simulink model "Test1_1"  (R2021a)
settings: Solver=FixedStepAuto  StartTime=0  StopTime=0.2  FixedStep=0.2  RelTol=1e-3
libraries: spsDistributedParametersLineLib x46, spsThreePhaseSeriesRLCLoadLib x15, spsThreePhaseVIMeasurementLib x3, spsGroundLib x1, spsThreePhaseSourceLib x1, spsSeriesRLCBranchLib x1, spspowerguiLib x1
settings Model: Creator=Admin  LastModifiedBy=Admin

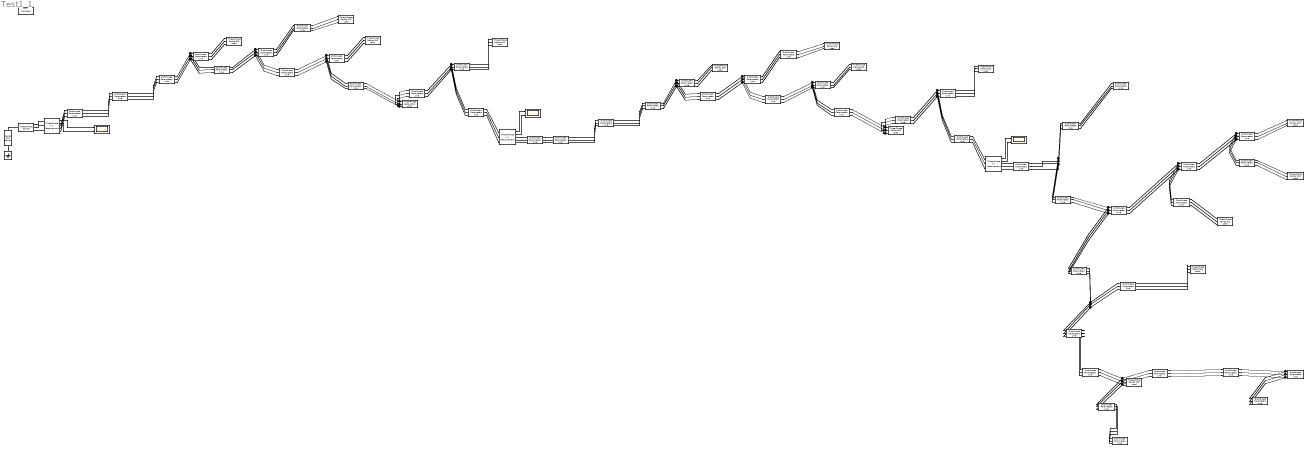
== system Test1_1 ==
  Ground : spsGroundLib/Ground  LConnTagsString=a
  Line 1 : spsDistributedParametersLineLib/Distributed Parameters Line  Phases=3  Length=0.24001  Frequency=50  Resistance=[0.646656091154803 0.0486237908083191 0.0486712220507153;0.0486237908083191 0.646561225344642 0.0486237934466192;0.0486712220507153 0.0486237934466192 0.646656091154803]  Inductance=[0.00282448912315926 0.00133270803418135 0.00132951476746136;0.00133270803418135 0.00282479813276775 0.00133799988507366;0.00132951476746136 0.00133799988507366 0.00282448912315926]  Capacitance=[7.89543174552926e-09 -1.85986777702161e-09 -1.7901190036642e-09;-1.85986777702161e-09 7.82540023894543e-09 -1.8957321828871e-09;-1.7901190036642e-09 -1.8957321828871e-09 7.91264394645417e-09]  x1=[156.806777459941 2289.04435554891 2292.85307010136;314.159265358979 314.159265358979 314.159265358979;1.01044698558813 -0.751410505261297 -2.32103514524067]  x2=[159.41925430945 1994.46757360395 1998.0250826666;314.159265358979 314.159265358979 314.159265358979;1.01620866542738 -0.846411494774192 -2.41545713049329]  x3=[6.24173255134266 1953.73927090339 1957.2720596961;314.159265358979 314.159265358979 314.159265358979;0.201344542731968 2.28105028050416 0.712425537947585]  x4=[6.05480721743813 1964.60242893867 1968.23812115216;314.159265358979 314.159265358979 314.159265358979;-2.97338155580937 -0.860183806246892 -2.42880992327048]  x5=1.1500013657538e-06  V1=ones(3,3)  V2=ones(3,3)  I1=ones(3,3)  I2=ones(3,3)  nHarmo=1  Measurements=None  Decoupling=off  VsMag0=0  VrMag0=0  VsAngle0=0  VrAngle0=0  IsMag0=0  IrMag0=0  IsAngle0=0  IrAngle0=0
      settings: SourceProductBaseCode=PS
  Line 10 : spsDistributedParametersLineLib/Distributed Parameters Line  Phases=3  Length=0.17  Frequency=50  Resistance=[0.646656091154803 0.0486237908083191 0.0486712220507153;0.0486237908083191 0.646561225344642 0.0486237934466192;0.0486712220507153 0.0486237934466192 0.646656091154803]  Inductance=[0.00282448912315926 0.00133270803418135 0.00132951476746136;0.00133270803418135 0.00282479813276775 0.00133799988507366;0.00132951476746136 0.00133799988507366 0.00282448912315926]  Capacitance=[7.89543174552926e-09 -1.85986777702161e-09 -1.7901190036642e-09;-1.85986777702161e-09 7.82540023894543e-09 -1.8957321828871e-09;-1.7901190036642e-09 -1.8957321828871e-09 7.91264394645417e-09]  x1=[137.717423229215 4738.81854218925 4741.80718996898;314.159265358979 314.159265358979 314.159265358979;0.961344854953636 -0.452365781969037 -2.02351010001284]  x2=[137.717927237638 4738.74941186832 4741.73816542518;314.159265358979 314.159265358979 314.159265358979;0.961345276145547 -0.452367573782606 -2.02351184606127]  x3=[0.121202473593997 11.5997833117508 11.6995568188445;314.159265358979 314.159265358979 314.159265358979;0.949832628337509 -0.42843606174828 -1.99977984923718]  x4=[0.119616166392622 12.521360958643 12.6220419925632;314.159265358979 314.159265358979 314.159265358979;0.972752580813695 -0.47473151222512 -2.04570347187694]  x5=8.14550361143895e-07  V1=ones(3,3)  V2=ones(3,3)  I1=ones(3,3)  I2=ones(3,3)  nHarmo=1  Measurements=None  Decoupling=off  VsMag0=0  VrMag0=0  VsAngle0=0  VrAngle0=0  IsMag0=0  IrMag0=0  IsAngle0=0  IrAngle0=0
      settings: SourceProductBaseCode=PS
  Line 11 : spsDistributedParametersLineLib/Distributed Parameters Line  Phases=3  Length=0.27999  Frequency=50  Resistance=[0.646656091154803 0.0486237908083191 0.0486712220507153;0.0486237908083191 0.646561225344642 0.0486237934466192;0.0486712220507153 0.0486237934466192 0.646656091154803]  Inductance=[0.00282448912315926 0.00133270803418135 0.00132951476746136;0.00133270803418135 0.00282479813276775 0.00133799988507366;0.00132951476746136 0.00133799988507366 0.00282448912315926]  Capacitance=[7.89543174552926e-09 -1.85986777702161e-09 -1.7901190036642e-09;-1.85986777702161e-09 7.82540023894543e-09 -1.8957321828871e-09;-1.7901190036642e-09 -1.8957321828871e-09 7.91264394645417e-09]  x1=[134.730981314477 5143.73431992549 5146.4499790882;314.159265358979 314.159265358979 314.159265358979;0.952121116671597 -0.431747792647745 -2.00297123761667]  x2=[137.717423229215 4738.81854218925 4741.80718996897;314.159265358979 314.159265358979 314.159265358979;0.96117928859628 -0.452497313565888 -2.02364175681846]  x3=[6.24015054861833 1949.40643992551 1952.88365407007;314.159265358979 314.159265358979 314.159265358979;0.19792740943073 2.27856091470476 0.70993208770443]  x4=[6.06948764855415 1972.37687159483 1976.07011587042;314.159265358979 314.159265358979 314.159265358979;-2.97066194767635 -0.857820676412098 -2.42644623491347]  x5=1.341564444804e-06  V1=ones(3,3)  V2=ones(3,3)  I1=ones(3,3)  I2=ones(3,3)  nHarmo=1  Measurements=None  Decoupling=off  VsMag0=0  VrMag0=0  VsAngle0=0  VrAngle0=0  IsMag0=0  IrMag0=0  IsAngle0=0  IrAngle0=0
      settings: SourceProductBaseCode=PS
  Line 12 : spsDistributedParametersLineLib/Distributed Parameters Line  Phases=3  Length=0.01  Frequency=50  Resistance=[0.646656091154803 0.0486237908083191 0.0486712220507153;0.0486237908083191 0.646561225344642 0.0486237934466192;0.0486712220507153 0.0486237934466192 0.646656091154803]  Inductance=[0.00282448912315926 0.00133270803418135 0.00132951476746136;0.00133270803418135 0.00282479813276775 0.00133799988507366;0.00132951476746136 0.00133799988507366 0.00282448912315926]  Capacitance=[7.89543174552926e-09 -1.85986777702161e-09 -1.7901190036642e-09;-1.85986777702161e-09 7.82540023894543e-09 -1.8957321828871e-09;-1.7901190036642e-09 -1.8957321828871e-09 7.91264394645417e-09]  x1=[134.624527579055 5158.23373249821 5160.93937939325;314.159265358979 314.159265358979 314.159265358979;0.952196584387825 -0.430744147583394 -2.00196980484842]  x2=[134.730981314477 5143.73431992549 5146.4499790882;314.159265358979 314.159265358979 314.159265358979;0.952527528716534 -0.431424924970376 -2.00264806259214]  x3=[6.24066120987054 1949.77580962925 1953.25644793354;314.159265358979 314.159265358979 314.159265358979;0.198319422837552 2.27887149292865 0.710242959177239]  x4=[6.07113450564641 1973.61885273018 1977.32373149217;314.159265358979 314.159265358979 314.159265358979;-2.96983216288509 -0.857163833200009 -2.42578877245703]  x5=4.79147271261115e-08  V1=ones(3,3)  V2=ones(3,3)  I1=ones(3,3)  I2=ones(3,3)  nHarmo=1  Measurements=None  Decoupling=off  VsMag0=0  VrMag0=0  VsAngle0=0  VrAngle0=0  IsMag0=0  IrMag0=0  IsAngle0=0  IrAngle0=0
      settings: SourceProductBaseCode=PS
  Line 13 : spsDistributedParametersLineLib/Distributed Parameters Line  Phases=3  Length=0.04  Frequency=50  Resistance=[0.646656091154803 0.0486237908083191 0.0486712220507153;0.0486237908083191 0.646561225344642 0.0486237934466192;0.0486712220507153 0.0486237934466192 0.646656091154803]  Inductance=[0.00282448912315926 0.00133270803418135 0.00132951476746136;0.00133270803418135 0.00282479813276775 0.00133799988507366;0.00132951476746136 0.00133799988507366 0.00282448912315926]  Capacitance=[7.89543174552926e-09 -1.85986777702161e-09 -1.7901190036642e-09;-1.85986777702161e-09 7.82540023894543e-09 -1.8957321828871e-09;-1.7901190036642e-09 -1.8957321828871e-09 7.91264394645417e-09]  x1=[134.198860362037 5216.25494933431 5218.9203856369;314.159265358979 314.159265358979 314.159265358979;0.950822400125934 -0.428094767615988 -1.9993303521305]  x2=[134.624527579055 5158.23373249821 5160.93937939325;314.159265358979 314.159265358979 314.159265358979;0.952151425821402 -0.430780023098491 -2.00200571451447]  x3=[6.24044022443603 1949.6120636545 1953.09117465905;314.159265358979 314.159265358979 314.159265358979;0.198214322239693 2.27878764327756 0.710159028664123]  x4=[6.07111576572209 1973.60352039945 1977.3082528197;314.159265358979 314.159265358979 314.159265358979;-2.96986211621341 -0.85718782340359 -2.42581278603856]  x5=1.91658908504446e-07  V1=ones(3,3)  V2=ones(3,3)  I1=ones(3,3)  I2=ones(3,3)  nHarmo=1  Measurements=None  Decoupling=off  VsMag0=0  VrMag0=0  VsAngle0=0  VrAngle0=0  IsMag0=0  IrMag0=0  IsAngle0=0  IrAngle0=0
      settings: SourceProductBaseCode=PS
  Line 2 : spsDistributedParametersLineLib/Distributed Parameters Line  Phases=3  Length=0.02  Frequency=50  Resistance=[0.646656091154803 0.0486237908083191 0.0486712220507153;0.0486237908083191 0.646561225344642 0.0486237934466192;0.0486712220507153 0.0486237934466192 0.646656091154803]  Inductance=[0.00282448912315926 0.00133270803418135 0.00132951476746136;0.00133270803418135 0.00282479813276775 0.00133799988507366;0.00132951476746136 0.00133799988507366 0.00282448912315926]  Capacitance=[7.89543174552926e-09 -1.85986777702161e-09 -1.7901190036642e-09;-1.85986777702161e-09 7.82540023894543e-09 -1.8957321828871e-09;-1.7901190036642e-09 -1.8957321828871e-09 7.91264394645417e-09]  x1=[156.806777459941 2289.04435554891 2292.85307010136;314.159265358979 314.159265358979 314.159265358979;1.01077816346141 -0.751147406192081 -2.32077179571977]  x2=[156.806785976177 2289.04321851652 2292.85193332345;314.159265358979 314.159265358979 314.159265358979;1.01077815828353 -0.751147536284466 -2.32077192407531]  x3=[0.13717054036225 5.75443719278579 5.80881227749304;314.159265358979 314.159265358979 314.159265358979;1.00918028356381 -0.745806305067407 -2.31547605369833]  x4=[0.137030436627376 5.89619014071261 5.95082798871036;314.159265358979 314.159265358979 314.159265358979;1.01234755059242 -0.756383856543157 -2.32596493554703]  x5=9.5829454252223e-08  V1=ones(3,3)  V2=ones(3,3)  I1=ones(3,3)  I2=ones(3,3)  nHarmo=1  Measurements=None  Decoupling=off  VsMag0=0  VrMag0=0  VsAngle0=0  VrAngle0=0  IsMag0=0  IrMag0=0  IsAngle0=0  IrAngle0=0
      settings: SourceProductBaseCode=PS
  Line 3 : spsDistributedParametersLineLib/Distributed Parameters Line  Phases=3  Length=0.5  Frequency=50  Resistance=[0.646656091154803 0.0486237908083191 0.0486712220507153;0.0486237908083191 0.646561225344642 0.0486237934466192;0.0486712220507153 0.0486237934466192 0.646656091154803]  Inductance=[0.00282448912315926 0.00133270803418135 0.00132951476746136;0.00133270803418135 0.00282479813276775 0.00133799988507366;0.00132951476746136 0.00133799988507366 0.00282448912315926]  Capacitance=[7.89543174552926e-09 -1.85986777702161e-09 -1.7901190036642e-09;-1.85986777702161e-09 7.82540023894543e-09 -1.8957321828871e-09;-1.7901190036642e-09 -1.8957321828871e-09 7.91264394645417e-09]  x1=[151.381670066741 2947.95085767605 2951.82529065523;314.159265358979 314.159265358979 314.159265358979;0.997415388913609 -0.617619917483095 -2.18800176165379]  x2=[156.806777459941 2289.04435554891 2292.85307010136;314.159265358979 314.159265358979 314.159265358979;1.01005562639866 -0.751721414433634 -2.32134635037653]  x3=[6.23941383066717 1951.93705204109 1955.45243536136;314.159265358979 314.159265358979 314.159265358979;0.200188858984882 2.28012943253653 0.711503799574193]  x4=[6.05546788002709 1965.0024474538 1968.64128594745;314.159265358979 314.159265358979 314.159265358979;-2.97342375138114 -0.860219461653461 -2.42884562437829]  x5=2.39573635630557e-06  V1=ones(3,3)  V2=ones(3,3)  I1=ones(3,3)  I2=ones(3,3)  nHarmo=1  Measurements=None  Decoupling=off  VsMag0=0  VrMag0=0  VsAngle0=0  VrAngle0=0  IsMag0=0  IrMag0=0  IsAngle0=0  IrAngle0=0
      settings: SourceProductBaseCode=PS
  Line 4 : spsDistributedParametersLineLib/Distributed Parameters Line  Phases=3  Length=0.23  Frequency=50  Resistance=[0.646656091154803 0.0486237908083191 0.0486712220507153;0.0486237908083191 0.646561225344642 0.0486237934466192;0.0486712220507153 0.0486237934466192 0.646656091154803]  Inductance=[0.00282448912315926 0.00133270803418135 0.00132951476746136;0.00133270803418135 0.00282479813276775 0.00133799988507366;0.00132951476746136 0.00133799988507366 0.00282448912315926]  Capacitance=[7.89543174552926e-09 -1.85986777702161e-09 -1.7901190036642e-09;-1.85986777702161e-09 7.82540023894543e-09 -1.8957321828871e-09;-1.7901190036642e-09 -1.8957321828871e-09 7.91264394645417e-09]  x1=[148.893866632266 3263.64496633825 3267.43134956967;314.159265358979 314.159265358979 314.159265358979;0.991698295023853 -0.574139543862195 -2.14474183596209]  x2=[151.381670066741 2947.95085767605 2951.82529065523;314.159265358979 314.159265358979 314.159265358979;0.997821816011403 -0.617297037847221 -2.18767857465937]  x3=[6.24075884536362 1952.25898948164 1955.77238425822;314.159265358979 314.159265358979 314.159265358979;0.200159169891873 2.2801199867809 0.711493977116933]  x4=[6.05971930332911 1967.50475507511 1971.16201304221;314.159265358979 314.159265358979 314.159265358979;-2.97234682394957 -0.859356129090504 -2.42798183096632]  x5=1.10203872390056e-06  V1=ones(3,3)  V2=ones(3,3)  I1=ones(3,3)  I2=ones(3,3)  nHarmo=1  Measurements=None  Decoupling=off  VsMag0=0  VrMag0=0  VsAngle0=0  VrAngle0=0  IsMag0=0  IrMag0=0  IsAngle0=0  IrAngle0=0
      settings: SourceProductBaseCode=PS
  Line 44 : spsDistributedParametersLineLib/Distributed Parameters Line  Phases=3  Length=1.1099  Frequency=50  Resistance=[0.502970710632245 0.0486237908083191 0.0486712220507153;0.0486237908083191 0.502875844822084 0.0486237934466192;0.0486712220507153 0.0486237934466192 0.502970710632245]  Inductance=[0.00286900545038753 0.00133270803418135 0.00132951476746136;0.00133270803418135 0.00286931445999602 0.00133799988507366;0.00132951476746136 0.00133799988507366 0.00286900545038753]  Capacitance=[8.11484299003193e-09 -1.94249816214699e-09 -1.86930692621136e-09;-1.94249816214699e-09 8.0425699231653e-09 -1.98049571960044e-09;-1.86930692621136e-09 -1.98049571960044e-09 8.13337738722527e-09]  x1=[176.041178073117 1994.09587758174 1997.08496491156;314.159265358979 314.159265358979 314.159265358979;0.937512580231571 -0.841595516654179 -2.41068590837705]  x2=[176.041429024076 1994.09774203895 1997.08683636866;314.159265358979 314.159265358979 314.159265358979;0.937512088108202 -0.841596394298114 -2.41068679358083]  x3=[0.154334056344399 5.07254983951833 5.11916023387305;314.159265358979 314.159265358979 314.159265358979;0.935823830196104 -0.84296342635579 -2.41205536081699]  x4=[0.15433405650098 5.0725498409922 5.11916023562135;314.159265358979 314.159265358979 314.159265358979;0.937512087880638 -0.84159639430282 -2.41068679356359]  x5=5.37467579168161e-06  V1=ones(3,3)  V2=ones(3,3)  I1=ones(3,3)  I2=ones(3,3)  nHarmo=1  Measurements=None  Decoupling=off  VsMag0=0  VrMag0=0  VsAngle0=0  VrAngle0=0  IsMag0=0  IrMag0=0  IsAngle0=0  IrAngle0=0
      settings: SourceProductBaseCode=PS
  Line 45 : spsDistributedParametersLineLib/Distributed Parameters Line  Phases=3  Length=0.03  Frequency=50  Resistance=[0.476003738225748 0.351747138225748 0.351747138225748;0.351747138225748 0.476003738225748 0.351747138225748;0.351747138225748 0.351747138225748 0.476003738225748]  Inductance=[0.000705954362986426 0.000459934243504405 0.000459934243504405;0.000459934243504405 0.000705954362986426 0.000459934243504405;0.000459934243504405 0.000459934243504405 0.000705954362986426]  Capacitance=[5.7561313269996e-07 -1.37543883484145e-07 -1.37543912800485e-07;-1.37543883484145e-07 5.75613027339387e-07 -1.37543875208088e-07;-1.37543912800485e-07 -1.37543875208088e-07 5.75613005057695e-07]  x1=[140.067507206974 1994.04557140135 1997.97862030497;314.159265358979 314.159265358979 314.159265358979;1.13103266143179 -0.764805817062905 -2.33393929024607]  x2=[140.067512372288 1994.04560306697 1997.97865212982;314.159265358979 314.159265358979 314.159265358979;1.13103254429501 -0.764805842557438 -2.33393931587598]  x3=[1.90359295650131 107.343811588221 107.55551404486;314.159265358979 314.159265358979 314.159265358979;1.13069546040223 -0.764995323142153 -2.33412939096158]  x4=[1.90368522741435 107.343794545186 107.555524609154;314.159265358979 314.159265358979 314.159265358979;1.13116138069285 -0.76474118135641 -2.33387406006431]  x5=6.63129528657629e-07  V1=ones(3,3)  V2=ones(3,3)  I1=ones(3,3)  I2=ones(3,3)  nHarmo=1  Measurements=None  Decoupling=off  VsMag0=0  VrMag0=0  VsAngle0=0  VrAngle0=0  IsMag0=0  IrMag0=0  IsAngle0=0  IrAngle0=0
      settings: SourceProductBaseCode=PS
  Line 46 : spsDistributedParametersLineLib/Distributed Parameters Line  Phases=3  Length=0.28002  Frequency=50  Resistance=[0.476003738225748 0.351747138225748 0.351747138225748;0.351747138225748 0.476003738225748 0.351747138225748;0.351747138225748 0.351747138225748 0.476003738225748]  Inductance=[0.000705954362986426 0.000459934243504405 0.000459934243504405;0.000459934243504405 0.000705954362986426 0.000459934243504405;0.000459934243504405 0.000459934243504405 0.000705954362986426]  Capacitance=[5.7561313269996e-07 -1.37543883484145e-07 -1.37543912800485e-07;-1.37543883484145e-07 5.75613027339387e-07 -1.37543875208088e-07;-1.37543912800485e-07 -1.37543875208088e-07 5.75613005057695e-07]  x1=[140.067507206974 1994.04557140135 1997.97862030497;314.159265358979 314.159265358979 314.159265358979;1.12929645349993 -0.765846222255273 -2.33497969535801]  x2=[140.067787182756 1994.04703476282 1997.98008719615;314.159265358979 314.159265358979 314.159265358979;1.12929162670007 -0.765847401848355 -2.33498087583294]  x3=[1.89789588728064 107.209321409248 107.420763113053;314.159265358979 314.159265358979 314.159265358979;1.12725437496433 -0.76705912034498 -2.33619301026011]  x4=[1.89796082095005 107.209309806491 107.420770208945;314.159265358979 314.159265358979 314.159265358979;1.12938694957278 -0.765800293242872 -2.33493335043468]  x5=6.18965102049031e-06  V1=ones(3,3)  V2=ones(3,3)  I1=ones(3,3)  I2=ones(3,3)  nHarmo=1  Measurements=None  Decoupling=off  VsMag0=0  VrMag0=0  VsAngle0=0  VrAngle0=0  IsMag0=0  IrMag0=0  IsAngle0=0  IrAngle0=0
      settings: SourceProductBaseCode=PS
  Line 47 : spsDistributedParametersLineLib/Distributed Parameters Line  Phases=3  Length=0.28002  Frequency=50  Resistance=[0.646656091154803 0.0486237908083191 0.0486712220507153;0.0486237908083191 0.646561225344642 0.0486237934466192;0.0486712220507153 0.0486237934466192 0.646656091154803]  Inductance=[0.00282448912315926 0.00133270803418135 0.00132951476746136;0.00133270803418135 0.00282479813276775 0.00133799988507366;0.00132951476746136 0.00133799988507366 0.00282448912315926]  Capacitance=[7.89543174552926e-09 -1.85986777702161e-09 -1.7901190036642e-09;-1.85986777702161e-09 7.82540023894543e-09 -1.8957321828871e-09;-1.7901190036642e-09 -1.8957321828871e-09 7.91264394645417e-09]  x1=[159.450836212371 1994.03630645724 1997.5930850958;314.159265358979 314.159265358979 314.159265358979;1.01609729305141 -0.846696591151605 -2.41574119338602]  x2=[159.450906639713 1994.03685996462 1997.59364061124;314.159265358979 314.159265358979 314.159265358979;1.01609710390738 -0.846696944332278 -2.4157415495164]  x3=[0.139394917805582 5.07298472412607 5.12105417855764;314.159265358979 314.159265358979 314.159265358979;1.01483976738527 -0.847693086082789 -2.41673856198392]  x4=[0.139394174108232 5.07298484806111 5.12105412073545;314.159265358979 314.159265358979 314.159265358979;1.01693310594968 -0.846035347146105 -2.41507939770091]  x5=1.34170818898537e-06  V1=ones(3,3)  V2=ones(3,3)  I1=ones(3,3)  I2=ones(3,3)  nHarmo=1  Measurements=None  Decoupling=off  VsMag0=0  VrMag0=0  VsAngle0=0  VrAngle0=0  IsMag0=0  IrMag0=0  IsAngle0=0  IrAngle0=0
      settings: SourceProductBaseCode=PS
  Line 48 : spsDistributedParametersLineLib/Distributed Parameters Line  Phases=3  Length=0.3  Frequency=50  Resistance=[0.80718830189013 0.0486237908083191 0.0486712220507153;0.0486237908083191 0.807093436079969 0.0486237934466192;0.0486712220507153 0.0486237934466192 0.80718830189013]  Inductance=[0.00279786707424938 0.00133270803418135 0.00132951476746136;0.00133270803418135 0.00279817608385787 0.00133799988507366;0.00132951476746136 0.00133799988507366 0.00279786707424938]  Capacitance=[7.73340098830622e-09 -1.79942827973291e-09 -1.73218055098733e-09;-1.79942827973291e-09 7.66505189233746e-09 -1.83375898618858e-09;-1.73218055098733e-09 -1.83375898618858e-09 7.749673531177e-09]  x1=[147.939133023316 1994.00252129492 1997.97662588148;314.159265358979 314.159265358979 314.159265358979;1.08434791512588 -0.850955285689131 -2.4199425962697]  x2=[147.939147884205 1994.00264447014 1997.97674951097;314.159265358979 314.159265358979 314.159265358979;1.08434786220581 -0.850955387187637 -2.41994269861345]  x3=[0.128901027196759 5.05947408132654 5.1081835056915;314.159265358979 314.159265358979 314.159265358979;1.08389966452075 -0.851306827100118 -2.42029443513027]  x4=[0.128901026894174 5.05947408128851 5.10818350470838;314.159265358979 314.159265358979 314.159265358979;1.08434786133197 -0.850955387242975 -2.41994269861003]  x5=1.42674452918375e-06  V1=ones(3,3)  V2=ones(3,3)  I1=ones(3,3)  I2=ones(3,3)  nHarmo=1  Measurements=None  Decoupling=off  VsMag0=0  VrMag0=0  VsAngle0=0  VrAngle0=0  IsMag0=0  IrMag0=0  IsAngle0=0  IrAngle0=0
      settings: SourceProductBaseCode=PS
  Line 49 : spsDistributedParametersLineLib/Distributed Parameters Line  Phases=3  Length=0.26  Frequency=50  Resistance=[0.646656091154803 0.0486237908083191 0.0486712220507153;0.0486237908083191 0.646561225344642 0.0486237934466192;0.0486712220507153 0.0486237934466192 0.646656091154803]  Inductance=[0.00282448912315926 0.00133270803418135 0.00132951476746136;0.00133270803418135 0.00282479813276775 0.00133799988507366;0.00132951476746136 0.00133799988507366 0.00282448912315926]  Capacitance=[7.89543174552926e-09 -1.85986777702161e-09 -1.7901190036642e-09;-1.85986777702161e-09 7.82540023894543e-09 -1.8957321828871e-09;-1.7901190036642e-09 -1.8957321828871e-09 7.91264394645417e-09]  x1=[159.450906639713 1994.03685996462 1997.59364061124;314.159265358979 314.159265358979 314.159265358979;1.01612723972403 -0.846673003405204 -2.41571758579925]  x2=[159.450918851672 1994.03695634835 1997.59373735104;314.159265358979 314.159265358979 314.159265358979;1.01612720669562 -0.8466730649035 -2.41571764781801]  x3=[0.139395866645988 5.07309981328857 5.12117114312411;314.159265358979 314.159265358979 314.159265358979;1.01573584725394 -0.846983955099221 -2.41602883408079]  x4=[0.139395866634972 5.07309981174401 5.12117114133114;314.159265358979 314.159265358979 314.159265358979;1.01612720842007 -0.846673065089804 -2.41571764765183]  x5=1.2457829052789e-06  V1=ones(3,3)  V2=ones(3,3)  I1=ones(3,3)  I2=ones(3,3)  nHarmo=1  Measurements=None  Decoupling=off  VsMag0=0  VrMag0=0  VsAngle0=0  VrAngle0=0  IsMag0=0  IrMag0=0  IsAngle0=0  IrAngle0=0
      settings: SourceProductBaseCode=PS
  Line 5 : spsDistributedParametersLineLib/Distributed Parameters Line  Phases=3  Length=1.62  Frequency=50  Resistance=[0.80718830189013 0.0486237908083191 0.0486712220507153;0.0486237908083191 0.807093436079969 0.0486237934466192;0.0486712220507153 0.0486237934466192 0.80718830189013]  Inductance=[0.00279786707424938 0.00133270803418135 0.00132951476746136;0.00133270803418135 0.00279817608385787 0.00133799988507366;0.00132951476746136 0.00133799988507366 0.00279786707424938]  Capacitance=[7.73340098830622e-09 -1.79942827973291e-09 -1.73218055098733e-09;-1.79942827973291e-09 7.66505189233746e-09 -1.83375898618858e-09;-1.73218055098733e-09 -1.83375898618858e-09 7.749673531177e-09]  x1=[125.888199100643 3263.65966141635 3267.79031196594;314.159265358979 314.159265358979 314.159265358979;1.07014406284904 -0.580039195774503 -2.15061989958838]  x2=[125.88865872902 3263.65855558813 3267.78922946379;314.159265358979 314.159265358979 314.159265358979;1.07014242225172 -0.580042000961513 -2.15062272408421]  x3=[0.109612775122241 8.2613178446553 8.33470841629561;314.159265358979 314.159265358979 314.159265358979;1.06747299264217 -0.58159829134088 -2.15218332448631]  x4=[0.109592728656291 8.26922562456906 8.34262765841689;314.159265358979 314.159265358979 314.159265358979;1.07039257279993 -0.580383016472921 -2.15096102526835]  x5=7.70442045759223e-06  V1=ones(3,3)  V2=ones(3,3)  I1=ones(3,3)  I2=ones(3,3)  nHarmo=1  Measurements=None  Decoupling=off  VsMag0=0  VrMag0=0  VsAngle0=0  VrAngle0=0  IsMag0=0  IrMag0=0  IsAngle0=0  IrAngle0=0
      settings: SourceProductBaseCode=PS
  Line 50 : spsDistributedParametersLineLib/Distributed Parameters Line  Phases=3  Length=0.02  Frequency=50  Resistance=[0.476003738225748 0.351747138225748 0.351747138225748;0.351747138225748 0.476003738225748 0.351747138225748;0.351747138225748 0.351747138225748 0.476003738225748]  Inductance=[0.000705954362986426 0.000459934243504405 0.000459934243504405;0.000459934243504405 0.000705954362986426 0.000459934243504405;0.000459934243504405 0.000459934243504405 0.000705954362986426]  Capacitance=[5.7561313269996e-07 -1.37543883484145e-07 -1.37543912800485e-07;-1.37543883484145e-07 5.75613027339387e-07 -1.37543875208088e-07;-1.37543912800485e-07 -1.37543875208088e-07 5.75613005057695e-07]  x1=[140.067461475806 1994.04572193785 1997.97877102815;314.159265358979 314.159265358979 314.159265358979;1.1311028945428 -0.764763926143592 -2.33389739917688]  x2=[140.067507206974 1994.04557140135 1997.97862030497;314.159265358979 314.159265358979 314.159265358979;1.13110210419364 -0.76476420418424 -2.33389767737062]  x3=[1.90379458359188 107.205560232195 107.416980727275;314.159265358979 314.159265358979 314.159265358979;1.12858679885131 -0.766052580413334 -2.33518706516769]  x4=[1.90395210493187 107.492988877227 107.705022727871;314.159265358979 314.159265358979 314.159265358979;1.13347910084245 -0.76356211258393 -2.33269457728375]  x5=4.42086352438419e-07  V1=ones(3,3)  V2=ones(3,3)  I1=ones(3,3)  I2=ones(3,3)  nHarmo=1  Measurements=None  Decoupling=off  VsMag0=0  VrMag0=0  VsAngle0=0  VrAngle0=0  IsMag0=0  IrMag0=0  IsAngle0=0  IrAngle0=0
      settings: SourceProductBaseCode=PS
  Line 51 : spsDistributedParametersLineLib/Distributed Parameters Line  Phases=3  Length=1.7101  Frequency=50  Resistance=[0.646656091154803 0.0486237908083191 0.0486712220507153;0.0486237908083191 0.646561225344642 0.0486237934466192;0.0486712220507153 0.0486237934466192 0.646656091154803]  Inductance=[0.00282448912315926 0.00133270803418135 0.00132951476746136;0.00133270803418135 0.00282479813276775 0.00133799988507366;0.00132951476746136 0.00133799988507366 0.00282448912315926]  Capacitance=[7.89543174552926e-09 -1.85986777702161e-09 -1.7901190036642e-09;-1.85986777702161e-09 7.82540023894543e-09 -1.8957321828871e-09;-1.7901190036642e-09 -1.8957321828871e-09 7.91264394645417e-09]  x1=[159.434216924154 1994.06687305595 1997.62429499923;314.159265358979 314.159265358979 314.159265358979;1.01397051629518 -0.848273829914017 -2.41732040176447]  x2=[159.450432897163 1994.03499301366 1997.59176799127;314.159265358979 314.159265358979 314.159265358979;1.01394953072372 -0.848405295765299 -2.4174515240815]  x3=[0.140424357868487 4.92335462242945 4.97106245663484;314.159265358979 314.159265358979 314.159265358979;0.976689775708697 -0.878406592183143 -2.44725440560169]  x4=[0.138339009885764 5.2101863624961 5.25832174536216;314.159265358979 314.159265358979 314.159265358979;1.04919801792014 -0.821918225205559 -2.39114198119224]  x5=8.19389748583632e-06  V1=ones(3,3)  V2=ones(3,3)  I1=ones(3,3)  I2=ones(3,3)  nHarmo=1  Measurements=None  Decoupling=off  VsMag0=0  VrMag0=0  VsAngle0=0  VrAngle0=0  IsMag0=0  IrMag0=0  IsAngle0=0  IrAngle0=0
      settings: SourceProductBaseCode=PS
  Line 52 : spsDistributedParametersLineLib/Distributed Parameters Line  Phases=3  Length=0.02  Frequency=50  Resistance=[0.646656091154803 0.0486237908083191 0.0486712220507153;0.0486237908083191 0.646561225344642 0.0486237934466192;0.0486712220507153 0.0486237934466192 0.646656091154803]  Inductance=[0.00282448912315926 0.00133270803418135 0.00132951476746136;0.00133270803418135 0.00282479813276775 0.00133799988507366;0.00132951476746136 0.00133799988507366 0.00282448912315926]  Capacitance=[7.89543174552926e-09 -1.85986777702161e-09 -1.7901190036642e-09;-1.85986777702161e-09 7.82540023894543e-09 -1.8957321828871e-09;-1.7901190036642e-09 -1.8957321828871e-09 7.91264394645417e-09]  x1=[159.434216924154 1994.06687305595 1997.62429499923;314.159265358979 314.159265358979 314.159265358979;1.01651459939881 -0.846252722978499 -2.41529737087826]  x2=[159.434233449095 1994.06437117717 1997.62179514991;314.159265358979 314.159265358979 314.159265358979;1.01651455261161 -0.846252753377473 -2.41529739765683]  x3=[0.13939024153263 4.94374785415629 4.99156990780943;314.159265358979 314.159265358979 314.159265358979;1.01303132944204 -0.826335458576535 -2.39554480562391]  x4=[0.139406554776425 5.20729050213767 5.25564996680037;314.159265358979 314.159265358979 314.159265358979;1.0199673106731 -0.865185186230515 -2.43408067605176]  x5=9.5829454252223e-08  V1=ones(3,3)  V2=ones(3,3)  I1=ones(3,3)  I2=ones(3,3)  nHarmo=1  Measurements=None  Decoupling=off  VsMag0=0  VrMag0=0  VsAngle0=0  VrAngle0=0  IsMag0=0  IrMag0=0  IsAngle0=0  IrAngle0=0
      settings: SourceProductBaseCode=PS
  Line 53 : spsDistributedParametersLineLib/Distributed Parameters Line  Phases=3  Length=0.02  Frequency=50  Resistance=[0.646656091154803 0.0486237908083191 0.0486712220507153;0.0486237908083191 0.646561225344642 0.0486237934466192;0.0486712220507153 0.0486237934466192 0.646656091154803]  Inductance=[0.00282448912315926 0.00133270803418135 0.00132951476746136;0.00133270803418135 0.00282479813276775 0.00133799988507366;0.00132951476746136 0.00133799988507366 0.00282448912315926]  Capacitance=[7.89543174552926e-09 -1.85986777702161e-09 -1.7901190036642e-09;-1.85986777702161e-09 7.82540023894543e-09 -1.8957321828871e-09;-1.7901190036642e-09 -1.8957321828871e-09 7.91264394645417e-09]  x1=[159.434004427504 1994.06969807982 1997.62712537534;314.159265358979 314.159265358979 314.159265358979;1.01651490874367 -0.846251123240228 -2.4152957785091]  x2=[159.434216924154 1994.06687305595 1997.62429499923;314.159265358979 314.159265358979 314.159265358979;1.01651459939881 -0.846252722978499 -2.41529737087826]  x3=[0.140550376835806 4.79918246505328 4.84679571886124;314.159265358979 314.159265358979 314.159265358979;0.975760126263114 -0.856708134290268 -2.42571661282824]  x4=[0.138479529171414 5.35045220808696 5.3990351748367;314.159265358979 314.159265358979 314.159265358979;1.05784884784109 -0.836895758448197 -2.40596509686568]  x5=9.5829454252223e-08  V1=ones(3,3)  V2=ones(3,3)  I1=ones(3,3)  I2=ones(3,3)  nHarmo=1  Measurements=None  Decoupling=off  VsMag0=0  VrMag0=0  VsAngle0=0  VrAngle0=0  IsMag0=0  IrMag0=0  IsAngle0=0  IrAngle0=0
      settings: SourceProductBaseCode=PS
  Line 54 : spsDistributedParametersLineLib/Distributed Parameters Line  Phases=3  Length=1.15  Frequency=50  Resistance=[0.646656091154803 0.0486237908083191 0.0486712220507153;0.0486237908083191 0.646561225344642 0.0486237934466192;0.0486712220507153 0.0486237934466192 0.646656091154803]  Inductance=[0.00282448912315926 0.00133270803418135 0.00132951476746136;0.00133270803418135 0.00282479813276775 0.00133799988507366;0.00132951476746136 0.00133799988507366 0.00282448912315926]  Capacitance=[7.89543174552926e-09 -1.85986777702161e-09 -1.7901190036642e-09;-1.85986777702161e-09 7.82540023894543e-09 -1.8957321828871e-09;-1.7901190036642e-09 -1.8957321828871e-09 7.91264394645417e-09]  x1=[159.434004427504 1994.06969807982 1997.62712537534;314.159265358979 314.159265358979 314.159265358979;1.01481393607513 -0.847602434308884 -2.41664837593021]  x2=[159.436593973299 1993.81619627619 1997.37383264922;314.159265358979 314.159265358979 314.159265358979;1.01480717385664 -0.847614516303686 -2.41666010492935]  x3=[0.139344375762193 4.82576502397844 4.87323625306902;314.159265358979 314.159265358979 314.159265358979;1.00461625069129 -0.815715661220324 -2.38506123462553]  x4=[0.139311518294218 5.31454729856164 5.36300293388667;314.159265358979 314.159265358979 314.159265358979;1.02327565800032 -0.877879729286988 -2.44667544350458]  x5=5.51019361950282e-06  V1=ones(3,3)  V2=ones(3,3)  I1=ones(3,3)  I2=ones(3,3)  nHarmo=1  Measurements=None  Decoupling=off  VsMag0=0  VrMag0=0  VsAngle0=0  VrAngle0=0  IsMag0=0  IrMag0=0  IsAngle0=0  IrAngle0=0
      settings: SourceProductBaseCode=PS
  Line 55 : spsDistributedParametersLineLib/Distributed Parameters Line  Phases=3  Length=0.18999  Frequency=50  Resistance=[0.646656091154803 0.0486237908083191 0.0486712220507153;0.0486237908083191 0.646561225344642 0.0486237934466192;0.0486712220507153 0.0486237934466192 0.646656091154803]  Inductance=[0.00282448912315926 0.00133270803418135 0.00132951476746136;0.00133270803418135 0.00282479813276775 0.00133799988507366;0.00132951476746136 0.00133799988507366 0.00282448912315926]  Capacitance=[7.89543174552926e-09 -1.85986777702161e-09 -1.7901190036642e-09;-1.85986777702161e-09 7.82540023894543e-09 -1.8957321828871e-09;-1.7901190036642e-09 -1.8957321828871e-09 7.91264394645417e-09]  x1=[159.436593973299 1993.81619627619 1997.37383264922;314.159265358979 314.159265358979 314.159265358979;1.01625226303498 -0.846466487862075 -2.41551098364595]  x2=[159.436702311302 1993.80079520723 1997.35844408271;314.159265358979 314.159265358979 314.159265358979;1.01625196060966 -0.846466741925637 -2.41551121551452]  x3=[0.139384682468638 4.98736902072087 5.03526752829464;314.159265358979 314.159265358979 314.159265358979;1.01372120639192 -0.833928109633916 -2.40307743341968]  x4=[0.139392398781965 5.15926374203587 5.20751177323792;314.159265358979 314.159265358979 314.159265358979;1.01849688704563 -0.858810775707692 -2.42775715887022]  x5=9.10331900668992e-07  V1=ones(3,3)  V2=ones(3,3)  I1=ones(3,3)  I2=ones(3,3)  nHarmo=1  Measurements=None  Decoupling=off  VsMag0=0  VrMag0=0  VsAngle0=0  VrAngle0=0  IsMag0=0  IrMag0=0  IsAngle0=0  IrAngle0=0
      settings: SourceProductBaseCode=PS
  Line 56 : spsDistributedParametersLineLib/Distributed Parameters Line  Phases=3  Length=0.34003  Frequency=50  Resistance=[0.646656091154803 0.0486237908083191 0.0486712220507153;0.0486237908083191 0.646561225344642 0.0486237934466192;0.0486712220507153 0.0486237934466192 0.646656091154803]  Inductance=[0.00282448912315926 0.00133270803418135 0.00132951476746136;0.00133270803418135 0.00282479813276775 0.00133799988507366;0.00132951476746136 0.00133799988507366 0.00282448912315926]  Capacitance=[7.89543174552926e-09 -1.85986777702161e-09 -1.7901190036642e-09;-1.85986777702161e-09 7.82540023894543e-09 -1.8957321828871e-09;-1.7901190036642e-09 -1.8957321828871e-09 7.91264394645417e-09]  x1=[159.436593973299 1993.81619627619 1997.37383264922;314.159265358979 314.159265358979 314.159265358979;1.01602640999145 -0.84664591327158 -2.41569057985574]  x2=[159.437062564447 1993.76799061169 1997.32566341844;314.159265358979 314.159265358979 314.159265358979;1.01602523094933 -0.846648511760201 -2.41569310928045]  x3=[0.139400669912724 4.91414204454292 4.96187584825958;314.159265358979 314.159265358979 314.159265358979;1.01009182155521 -0.826621601952847 -2.39584785255987]  x4=[0.13936006934663 5.23183524784472 5.28020744458036;314.159265358979 314.159265358979 314.159265358979;1.02144960313956 -0.865850983748701 -2.43473413484308]  x5=1.62924446646917e-06  V1=ones(3,3)  V2=ones(3,3)  I1=ones(3,3)  I2=ones(3,3)  nHarmo=1  Measurements=None  Decoupling=off  VsMag0=0  VrMag0=0  VsAngle0=0  VrAngle0=0  IsMag0=0  IrMag0=0  IsAngle0=0  IrAngle0=0
      settings: SourceProductBaseCode=PS
  Line 57 : spsDistributedParametersLineLib/Distributed Parameters Line  Phases=3  Length=0.12001  Frequency=50  Resistance=[0.646656091154803 0.0486237908083191 0.0486712220507153;0.0486237908083191 0.646561225344642 0.0486237934466192;0.0486712220507153 0.0486237934466192 0.646656091154803]  Inductance=[0.00282448912315926 0.00133270803418135 0.00132951476746136;0.00133270803418135 0.00282479813276775 0.00133799988507366;0.00132951476746136 0.00133799988507366 0.00282448912315926]  Capacitance=[7.89543174552926e-09 -1.85986777702161e-09 -1.7901190036642e-09;-1.85986777702161e-09 7.82540023894543e-09 -1.8957321828871e-09;-1.7901190036642e-09 -1.8957321828871e-09 7.91264394645417e-09]  x1=[159.437062564447 1993.76799061169 1997.32566341844;314.159265358979 314.159265358979 314.159265358979;1.01635642387546 -0.846385400732479 -2.41542974778966]  x2=[159.437106008724 1993.76195103605 1997.31962792097;314.159265358979 314.159265358979 314.159265358979;1.0163563170562 -0.846385647066924 -2.41542998503225]  x3=[0.13940038203012 5.01800388931349 5.0659738789957;314.159265358979 314.159265358979 314.159265358979;1.0147792997226 -0.839151877875453 -2.4082568428009]  x4=[0.139386471761622 5.12869741927316 5.17688981638374;314.159265358979 314.159265358979 314.159265358979;1.01775293673402 -0.853605013980352 -2.42259132217258]  x5=5.75024640240464e-07  V1=ones(3,3)  V2=ones(3,3)  I1=ones(3,3)  I2=ones(3,3)  nHarmo=1  Measurements=None  Decoupling=off  VsMag0=0  VrMag0=0  VsAngle0=0  VrAngle0=0  IsMag0=0  IrMag0=0  IsAngle0=0  IrAngle0=0
      settings: SourceProductBaseCode=PS
  Line 58 : spsDistributedParametersLineLib/Distributed Parameters Line  Phases=3  Length=0.82  Frequency=50  Resistance=[0.646656091154803 0.0486237908083191 0.0486712220507153;0.0486237908083191 0.646561225344642 0.0486237934466192;0.0486712220507153 0.0486237934466192 0.646656091154803]  Inductance=[0.00282448912315926 0.00133270803418135 0.00132951476746136;0.00133270803418135 0.00282479813276775 0.00133799988507366;0.00132951476746136 0.00133799988507366 0.00282448912315926]  Capacitance=[7.89543174552926e-09 -1.85986777702161e-09 -1.7901190036642e-09;-1.85986777702161e-09 7.82540023894543e-09 -1.8957321828871e-09;-1.7901190036642e-09 -1.8957321828871e-09 7.91264394645417e-09]  x1=[159.437062564447 1993.76799061169 1997.32566341844;314.159265358979 314.159265358979 314.159265358979;1.01530273904515 -0.847222484126239 -2.41626762802754]  x2=[159.437706153745 1993.69151082522 1997.24923810222;314.159265358979 314.159265358979 314.159265358979;1.01530113843963 -0.847226112780651 -2.41627114416478]  x3=[0.139360134005731 4.96605307651685 5.0138551124477;314.159265358979 314.159265358979 314.159265358979;1.01145645202668 -0.834305807817629 -2.4034668358605]  x4=[0.139333448291842 5.17297945479898 5.22119573941466;314.159265358979 314.159265358979 314.159265358979;1.01791354532471 -0.860587285688457 -2.42952584494006]  x5=3.92900762434114e-06  V1=ones(3,3)  V2=ones(3,3)  I1=ones(3,3)  I2=ones(3,3)  nHarmo=1  Measurements=None  Decoupling=off  VsMag0=0  VrMag0=0  VsAngle0=0  VrAngle0=0  IsMag0=0  IrMag0=0  IsAngle0=0  IrAngle0=0
      settings: SourceProductBaseCode=PS
  Line 59 : spsDistributedParametersLineLib/Distributed Parameters Line  Phases=3  Length=1.11  Frequency=50  Resistance=[0.646656091154803 0.0486237908083191 0.0486712220507153;0.0486237908083191 0.646561225344642 0.0486237934466192;0.0486712220507153 0.0486237934466192 0.646656091154803]  Inductance=[0.00282448912315926 0.00133270803418135 0.00132951476746136;0.00133270803418135 0.00282479813276775 0.00133799988507366;0.00132951476746136 0.00133799988507366 0.00282448912315926]  Capacitance=[7.89543174552926e-09 -1.85986777702161e-09 -1.7901190036642e-09;-1.85986777702161e-09 7.82540023894543e-09 -1.8957321828871e-09;-1.7901190036642e-09 -1.8957321828871e-09 7.91264394645417e-09]  x1=[159.419254310559 1994.4675734855 1998.0250825481;314.159265358979 314.159265358979 314.159265358979;1.01489908205575 -0.847451872798863 -2.41649849888386]  x2=[159.434004427504 1994.06969807982 1997.62712537534;314.159265358979 314.159265358979 314.159265358979;1.01487414749703 -0.847554600288755 -2.41660049637548]  x3=[0.140556500081023 4.55016802521499 4.59717276935351;314.159265358979 314.159265358979 314.159265358979;0.962381314678809 -0.826124355196915 -2.39546271669936]  x4=[0.138455551958621 5.58938103722576 5.63833276493993;314.159265358979 314.159265358979 314.159265358979;1.06650550532341 -0.866111225468013 -2.43494846728214]  x5=5.31853471099837e-06  V1=ones(3,3)  V2=ones(3,3)  I1=ones(3,3)  I2=ones(3,3)  nHarmo=1  Measurements=None  Decoupling=off  VsMag0=0  VrMag0=0  VsAngle0=0  VrAngle0=0  IsMag0=0  IrMag0=0  IsAngle0=0  IrAngle0=0
      settings: SourceProductBaseCode=PS
  Line 6 : spsDistributedParametersLineLib/Distributed Parameters Line  Phases=3  Length=0.54002  Frequency=50  Resistance=[0.646656091154803 0.0486237908083191 0.0486712220507153;0.0486237908083191 0.646561225344642 0.0486237934466192;0.0486712220507153 0.0486237934466192 0.646656091154803]  Inductance=[0.00282448912315926 0.00133270803418135 0.00132951476746136;0.00133270803418135 0.00282479813276775 0.00133799988507366;0.00132951476746136 0.00133799988507366 0.00282448912315926]  Capacitance=[7.89543174552926e-09 -1.85986777702161e-09 -1.7901190036642e-09;-1.85986777702161e-09 7.82540023894543e-09 -1.8957321828871e-09;-1.7901190036642e-09 -1.8957321828871e-09 7.91264394645417e-09]  x1=[143.075564008337 4022.40983924515 4025.83828253699;314.159265358979 314.159265358979 314.159265358979;0.976020045897074 -0.500200416639864 -2.07114942176074]  x2=[148.893866632266 3263.64496633825 3267.43134956967;314.159265358979 314.159265358979 314.159265358979;0.991231626398454 -0.574510281435208 -2.14511292645102]  x3=[6.23820594895896 1950.18981590391 1953.68388750545;314.159265358979 314.159265358979 314.159265358979;0.198848263808989 2.27910939508097 0.710482471111555]  x4=[6.06027373796471 1967.72576691583 1971.38505732425;314.159265358979 314.159265358979 314.159265358979;-2.97249972285949 -0.859445496613823 -2.42807123343329]  x5=2.58749109426427e-06  V1=ones(3,3)  V2=ones(3,3)  I1=ones(3,3)  I2=ones(3,3)  nHarmo=1  Measurements=None  Decoupling=off  VsMag0=0  VrMag0=0  VsAngle0=0  VrAngle0=0  IsMag0=0  IrMag0=0  IsAngle0=0  IrAngle0=0
      settings: SourceProductBaseCode=PS
  Line 60 : spsDistributedParametersLineLib/Distributed Parameters Line  Phases=3  Length=0.20998  Frequency=50  Resistance=[0.646656091154803 0.0486237908083191 0.0486712220507153;0.0486237908083191 0.646561225344642 0.0486237934466192;0.0486712220507153 0.0486237934466192 0.646656091154803]  Inductance=[0.00282448912315926 0.00133270803418135 0.00132951476746136;0.00133270803418135 0.00282479813276775 0.00133799988507366;0.00132951476746136 0.00133799988507366 0.00282448912315926]  Capacitance=[7.89543174552926e-09 -1.85986777702161e-09 -1.7901190036642e-09;-1.85986777702161e-09 7.82540023894543e-09 -1.8957321828871e-09;-1.7901190036642e-09 -1.8957321828871e-09 7.91264394645417e-09]  x1=[159.419254310559 1994.4675734855 1998.0250825481;314.159265358979 314.159265358979 314.159265358979;1.01652508247232 -0.846160122260372 -2.41520551869033]  x2=[159.733034103855 1959.34815012485 1962.86056264333;314.159265358979 314.159265358979 314.159265358979;1.01693000879211 -0.859919844540877 -2.4288792381102]  x3=[5.81368882645404 1954.7575240747 1958.21418010732;314.159265358979 314.159265358979 314.159265358979;0.0758207513055684 2.28142414704698 0.712799108344841]  x4=[5.65381092262754 1964.8187133012 1968.37080091939;314.159265358979 314.159265358979 314.159265358979;-3.10566497589273 -0.860131781432291 -2.42875848813043]  x5=1.42814635672088e-07  V1=ones(3,3)  V2=ones(3,3)  I1=ones(3,3)  I2=ones(3,3)  nHarmo=1  Measurements=None  Decoupling=off  VsMag0=0  VrMag0=0  VsAngle0=0  VrAngle0=0  IsMag0=0  IrMag0=0  IsAngle0=0  IrAngle0=0
      settings: SourceProductBaseCode=PS
  Line 61 : spsDistributedParametersLineLib/Distributed Parameters Line  Phases=3  Length=0.23002  Frequency=50  Resistance=[0.476003738225748 0.351747138225748 0.351747138225748;0.351747138225748 0.476003738225748 0.351747138225748;0.351747138225748 0.351747138225748 0.476003738225748]  Inductance=[0.000705954362986426 0.000459934243504405 0.000459934243504405;0.000459934243504405 0.000705954362986426 0.000459934243504405;0.000459934243504405 0.000459934243504405 0.000705954362986426]  Capacitance=[5.7561313269996e-07 -1.37543883484145e-07 -1.37543912800485e-07;-1.37543883484145e-07 5.75613027339387e-07 -1.37543875208088e-07;-1.37543912800485e-07 -1.37543875208088e-07 5.75613005057695e-07]  x1=[140.923088989266 1959.35938406052 1963.25737802957;314.159265358979 314.159265358979 314.159265358979;1.12938776250256 -0.77916863174631 -2.34822032842924]  x2=[140.923268767317 1959.36028163562 1963.25827739019;314.159265358979 314.159265358979 314.159265358979;1.12938481652344 -0.779169368217606 -2.34822106490041]  x3=[1.91066836601915 105.370820930055 105.580439877023;314.159265358979 314.159265358979 314.159265358979;1.12778896709952 -0.780126179418249 -2.34917787602386]  x4=[1.91066836831086 105.370820948731 105.580439895595;314.159265358979 314.159265358979 314.159265358979;1.12938481652402 -0.779169368216618 -2.34822106490251]  x5=5.08443513939426e-06  V1=ones(3,3)  V2=ones(3,3)  I1=ones(3,3)  I2=ones(3,3)  nHarmo=1  Measurements=None  Decoupling=off  VsMag0=0  VrMag0=0  VsAngle0=0  VrAngle0=0  IsMag0=0  IrMag0=0  IsAngle0=0  IrAngle0=0
      settings: SourceProductBaseCode=PS
  Line 62 : spsDistributedParametersLineLib/Distributed Parameters Line  Phases=3  Length=0.24  Frequency=50  Resistance=[0.646656091154803 0.0486237908083191 0.0486712220507153;0.0486237908083191 0.646561225344642 0.0486237934466192;0.0486712220507153 0.0486237934466192 0.646656091154803]  Inductance=[0.00282448912315926 0.00133270803418135 0.00132951476746136;0.00133270803418135 0.00282479813276775 0.00133799988507366;0.00132951476746136 0.00133799988507366 0.00282448912315926]  Capacitance=[7.89543174552926e-09 -1.85986777702161e-09 -1.7901190036642e-09;-1.85986777702161e-09 7.82540023894543e-09 -1.8957321828871e-09;-1.7901190036642e-09 -1.8957321828871e-09 7.91264394645417e-09]  x1=[131.891592747009 5565.19808455142 5567.63219452418;314.159265358979 314.159265358979 314.159265358979;0.943117828875783 -0.41341252510975 -1.98470450569848]  x2=[134.198860361112 5216.25494947947 5218.9203857818;314.159265358979 314.159265358979 314.159265358979;0.950521343014733 -0.428333937710009 -1.99956974989749]  x3=[5.65919040397014 1948.9656639006 1952.50013320203;314.159265358979 314.159265358979 314.159265358979;0.200649339611077 2.27801510380019 0.709338881017019]  x4=[5.49062351302118 1973.78455753586 1977.55185849412;314.159265358979 314.159265358979 314.159265358979;-2.96970298234479 -0.857623098119769 -2.42629492795019]  x5=1.14995345102668e-06  V1=ones(3,3)  V2=ones(3,3)  I1=ones(3,3)  I2=ones(3,3)  nHarmo=1  Measurements=None  Decoupling=off  VsMag0=0  VrMag0=0  VsAngle0=0  VrAngle0=0  IsMag0=0  IrMag0=0  IsAngle0=0  IrAngle0=0
      settings: SourceProductBaseCode=PS
  Line 63 : spsDistributedParametersLineLib/Distributed Parameters Line  Phases=3  Length=0.02  Frequency=50  Resistance=[0.646656091154803 0.0486237908083191 0.0486712220507153;0.0486237908083191 0.646561225344642 0.0486237934466192;0.0486712220507153 0.0486237934466192 0.646656091154803]  Inductance=[0.00282448912315926 0.00133270803418135 0.00132951476746136;0.00133270803418135 0.00282479813276775 0.00133799988507366;0.00132951476746136 0.00133799988507366 0.00282448912315926]  Capacitance=[7.89543174552926e-09 -1.85986777702161e-09 -1.7901190036642e-09;-1.85986777702161e-09 7.82540023894543e-09 -1.8957321828871e-09;-1.7901190036642e-09 -1.8957321828871e-09 7.91264394645417e-09]  x1=[131.891592747009 5565.19808455142 5567.63219452418;314.159265358979 314.159265358979 314.159265358979;0.943448991696207 -0.413149437999038 -1.98444116814747]  x2=[131.891601318725 5565.19689634062 5567.63100834352;314.159265358979 314.159265358979 314.159265358979;0.943449002989283 -0.413149464149948 -1.98444119362709]  x3=[0.11544346831214 14.0952153332801 14.2101767136837;314.159265358979 314.159265358979 314.159265358979;0.941751977798148 -0.410270065369696 -1.98158498689422]  x4=[0.115189481907542 14.2298888678593 14.3449576562899;314.159265358979 314.159265358979 314.159265358979;0.945119619566691 -0.416025389831499 -1.98729436636004]  x5=9.5829454252223e-08  V1=ones(3,3)  V2=ones(3,3)  I1=ones(3,3)  I2=ones(3,3)  nHarmo=1  Measurements=None  Decoupling=off  VsMag0=0  VrMag0=0  VsAngle0=0  VrAngle0=0  IsMag0=0  IrMag0=0  IsAngle0=0  IrAngle0=0
      settings: SourceProductBaseCode=PS
  Line 64 : spsDistributedParametersLineLib/Distributed Parameters Line  Phases=3  Length=0.5  Frequency=50  Resistance=[0.646656091154803 0.0486237908083191 0.0486712220507153;0.0486237908083191 0.646561225344642 0.0486237934466192;0.0486712220507153 0.0486237934466192 0.646656091154803]  Inductance=[0.00282448912315926 0.00133270803418135 0.00132951476746136;0.00133270803418135 0.00282479813276775 0.00133799988507366;0.00132951476746136 0.00133799988507366 0.00282448912315926]  Capacitance=[7.89543174552926e-09 -1.85986777702161e-09 -1.7901190036642e-09;-1.85986777702161e-09 7.82540023894543e-09 -1.8957321828871e-09;-1.7901190036642e-09 -1.8957321828871e-09 7.91264394645417e-09]  x1=[127.10903104861 6295.48950435492 6297.41893875871;314.159265358979 314.159265358979 314.159265358979;0.926441483086452 -0.387963501114633 -1.9593475206382]  x2=[131.891592747009 5565.19808455142 5567.63219452418;314.159265358979 314.159265358979 314.159265358979;0.942726454633463 -0.413723446240591 -1.98501572280422]  x3=[5.65712619641101 1947.16788071898 1950.68481854773;314.159265358979 314.159265358979 314.159265358979;0.199498822245796 2.27710033367642 0.708423140357235]  x4=[5.49125956278752 1974.18727249294 1977.95761633504;314.159265358979 314.159265358979 314.159265358979;-2.96973965138673 -0.857652333140068 -2.42632428239273]  x5=2.39573635630557e-06  V1=ones(3,3)  V2=ones(3,3)  I1=ones(3,3)  I2=ones(3,3)  nHarmo=1  Measurements=None  Decoupling=off  VsMag0=0  VrMag0=0  VsAngle0=0  VrAngle0=0  IsMag0=0  IrMag0=0  IsAngle0=0  IrAngle0=0
      settings: SourceProductBaseCode=PS
  Line 65 : spsDistributedParametersLineLib/Distributed Parameters Line  Phases=3  Length=0.23  Frequency=50  Resistance=[0.646656091154803 0.0486237908083191 0.0486712220507153;0.0486237908083191 0.646561225344642 0.0486237934466192;0.0486712220507153 0.0486237934466192 0.646656091154803]  Inductance=[0.00282448912315926 0.00133270803418135 0.00132951476746136;0.00133270803418135 0.00282479813276775 0.00133799988507366;0.00132951476746136 0.00133799988507366 0.00282448912315926]  Capacitance=[7.89543174552926e-09 -1.85986777702161e-09 -1.7901190036642e-09;-1.85986777702161e-09 7.82540023894543e-09 -1.8957321828871e-09;-1.7901190036642e-09 -1.8957321828871e-09 7.91264394645417e-09]  x1=[124.919285738109 6632.8469620951 6634.53616828906;314.159265358979 314.159265358979 314.159265358979;0.918932285202401 -0.377685065848571 -1.94910250658809]  x2=[127.10903104861 6295.48950435492 6297.41893875871;314.159265358979 314.159265358979 314.159265358979;0.926847910184245 -0.38764062147876 -1.95902433364378]  x3=[5.66119656832682 1948.3621408699 1951.87768959562;314.159265358979 314.159265358979 314.159265358979;0.199581126082684 2.27728031150108 0.708601142671808]  x4=[5.49794580883953 1977.57103823852 1981.36054639333;314.159265358979 314.159265358979 314.159265358979;-2.96853493163592 -0.856607463616824 -2.42528054555115]  x5=1.10203872390056e-06  V1=ones(3,3)  V2=ones(3,3)  I1=ones(3,3)  I2=ones(3,3)  nHarmo=1  Measurements=None  Decoupling=off  VsMag0=0  VrMag0=0  VsAngle0=0  VrAngle0=0  IsMag0=0  IrMag0=0  IsAngle0=0  IrAngle0=0
      settings: SourceProductBaseCode=PS
  Line 66 : spsDistributedParametersLineLib/Distributed Parameters Line  Phases=3  Length=1.62  Frequency=50  Resistance=[0.80718830189013 0.0486237908083191 0.0486712220507153;0.0486237908083191 0.807093436079969 0.0486237934466192;0.0486712220507153 0.0486237934466192 0.80718830189013]  Inductance=[0.00279786707424938 0.00133270803418135 0.00132951476746136;0.00133270803418135 0.00279817608385787 0.00133799988507366;0.00132951476746136 0.00133799988507366 0.00279786707424938]  Capacitance=[7.73340098830622e-09 -1.79942827973291e-09 -1.73218055098733e-09;-1.79942827973291e-09 7.66505189233746e-09 -1.83375898618858e-09;-1.73218055098733e-09 -1.83375898618858e-09 7.749673531177e-09]  x1=[73.8952918230876 6632.89366163882 6634.76575388419;314.159265358979 314.159265358979 314.159265358979;1.01444231795329 -0.383614285015778 -1.95499867923716]  x2=[73.8955979210801 6632.89810332107 6634.77022276576;314.159265358979 314.159265358979 314.159265358979;1.01444151065152 -0.383617665782324 -1.95500208086373]  x3=[0.0643644897980278 16.7924733580382 16.9249929532736;314.159265358979 314.159265358979 314.159265358979;1.01175529955734 -0.385451732868572 -1.95683827879511]  x4=[0.0643072933144445 16.8033749925563 16.9358996226528;314.159265358979 314.159265358979 314.159265358979;1.01470865520705 -0.383680322464446 -1.95506419841532]  x5=7.70442045759223e-06  V1=ones(3,3)  V2=ones(3,3)  I1=ones(3,3)  I2=ones(3,3)  nHarmo=1  Measurements=None  Decoupling=off  VsMag0=0  VrMag0=0  VsAngle0=0  VrAngle0=0  IsMag0=0  IrMag0=0  IsAngle0=0  IrAngle0=0
      settings: SourceProductBaseCode=PS
  Line 67 : spsDistributedParametersLineLib/Distributed Parameters Line  Phases=3  Length=0.54002  Frequency=50  Resistance=[0.646656091154803 0.0486237908083191 0.0486712220507153;0.0486237908083191 0.646561225344642 0.0486237934466192;0.0486712220507153 0.0486237934466192 0.646656091154803]  Inductance=[0.00282448912315926 0.00133270803418135 0.00132951476746136;0.00133270803418135 0.00282479813276775 0.00133799988507366;0.00132951476746136 0.00133799988507366 0.00282448912315926]  Capacitance=[7.89543174552926e-09 -1.85986777702161e-09 -1.7901190036642e-09;-1.85986777702161e-09 7.82540023894543e-09 -1.8957321828871e-09;-1.7901190036642e-09 -1.8957321828871e-09 7.91264394645417e-09]  x1=[119.810283207196 7427.11552101013 7428.22674768885;314.159265358979 314.159265358979 314.159265358979;0.898748119888331 -0.358239656935962 -1.92972147527054]  x2=[124.919285738109 6632.8469620951 6634.53616828906;314.159265358979 314.159265358979 314.159265358979;0.918465616577003 -0.378055803421584 -1.94947359707702]  x3=[5.6588530239754 1946.28244298577 1949.77857780318;314.159265358979 314.159265358979 314.159265358979;0.198272154714595 2.27627613384474 0.707596084817765]  x4=[5.49842005157672 1977.78036393304 1981.57183834624;314.159265358979 314.159265358979 314.159265358979;-2.9686859322517 -0.856689833755106 -2.42536291230108]  x5=2.58749109426427e-06  V1=ones(3,3)  V2=ones(3,3)  I1=ones(3,3)  I2=ones(3,3)  nHarmo=1  Measurements=None  Decoupling=off  VsMag0=0  VrMag0=0  VsAngle0=0  VrAngle0=0  IsMag0=0  IrMag0=0  IsAngle0=0  IrAngle0=0
      settings: SourceProductBaseCode=PS
  Line 68 : spsDistributedParametersLineLib/Distributed Parameters Line  Phases=3  Length=0.13998  Frequency=50  Resistance=[0.646656091154803 0.0486237908083191 0.0486712220507153;0.0486237908083191 0.646561225344642 0.0486237934466192;0.0486712220507153 0.0486237934466192 0.646656091154803]  Inductance=[0.00282448912315926 0.00133270803418135 0.00132951476746136;0.00133270803418135 0.00282479813276775 0.00133799988507366;0.00132951476746136 0.00133799988507366 0.00282448912315926]  Capacitance=[7.89543174552926e-09 -1.85986777702161e-09 -1.7901190036642e-09;-1.85986777702161e-09 7.82540023894543e-09 -1.8957321828871e-09;-1.7901190036642e-09 -1.8957321828871e-09 7.91264394645417e-09]  x1=[119.810283207196 7427.11552101013 7428.22674768885;314.159265358979 314.159265358979 314.159265358979;0.899350294318706 -0.357761268900648 -1.92924263184369]  x2=[119.810749669987 7427.05653665207 7428.16778288595;314.159265358979 314.159265358979 314.159265358979;0.899353152322059 -0.35776679797135 -1.9292481245871]  x3=[0.10665491486899 18.2242192642151 18.3719533542319;314.159265358979 314.159265358979 314.159265358979;0.888789173279573 -0.355702102669598 -1.92721121585688]  x4=[0.102851733737069 19.5720613607623 19.7202750190609;314.159265358979 314.159265358979 314.159265358979;0.910090252615542 -0.359845607715396 -1.93130229501859]  x5=6.70710350311308e-07  V1=ones(3,3)  V2=ones(3,3)  I1=ones(3,3)  I2=ones(3,3)  nHarmo=1  Measurements=None  Decoupling=off  VsMag0=0  VrMag0=0  VsAngle0=0  VrAngle0=0  IsMag0=0  IrMag0=0  IsAngle0=0  IrAngle0=0
      settings: SourceProductBaseCode=PS
  Line 69 : spsDistributedParametersLineLib/Distributed Parameters Line  Phases=3  Length=0.14997  Frequency=50  Resistance=[0.476003738225748 0.351747138225748 0.351747138225748;0.351747138225748 0.476003738225748 0.351747138225748;0.351747138225748 0.351747138225748 0.476003738225748]  Inductance=[0.000705954362986426 0.000459934243504405 0.000459934243504405;0.000459934243504405 0.000705954362986426 0.000459934243504405;0.000459934243504405 0.000459934243504405 0.000705954362986426]  Capacitance=[5.7561313269996e-07 -1.37543883484145e-07 -1.37543912800485e-07;-1.37543883484145e-07 5.75613027339387e-07 -1.37543875208088e-07;-1.37543912800485e-07 -1.37543875208088e-07 5.75613005057695e-07]  x1=[24.0560164851616 7428.15488535811 7429.2319451262;314.159265358979 314.159265358979 314.159265358979;1.14740326971435 -0.276568410078834 -1.84791591551979]  x2=[24.0560295312866 7428.14040816755 7429.21746583627;314.159265358979 314.159265358979 314.159265358979;1.14740201755767 -0.276569046969294 -1.84791655241019]  x3=[0.326470984193716 398.959396349274 399.017213369376;314.159265358979 314.159265358979 314.159265358979;1.14636125460116 -0.276466734510254 -1.84781423983873]  x4=[0.326470963273406 400.306093010476 400.364105294422;314.159265358979 314.159265358979 314.159265358979;1.14740197357211 -0.277293554287286 -1.84864105979185]  x5=3.31498451375949e-06  V1=ones(3,3)  V2=ones(3,3)  I1=ones(3,3)  I2=ones(3,3)  nHarmo=1  Measurements=None  Decoupling=off  VsMag0=0  VrMag0=0  VsAngle0=0  VrAngle0=0  IsMag0=0  IrMag0=0  IsAngle0=0  IrAngle0=0
      settings: SourceProductBaseCode=PS
  Line 7 : spsDistributedParametersLineLib/Distributed Parameters Line  Phases=3  Length=0.13998  Frequency=50  Resistance=[0.646656091154803 0.0486237908083191 0.0486712220507153;0.0486237908083191 0.646561225344642 0.0486237934466192;0.0486712220507153 0.0486237934466192 0.646656091154803]  Inductance=[0.00282448912315926 0.00133270803418135 0.00132951476746136;0.00133270803418135 0.00282479813276775 0.00133799988507366;0.00132951476746136 0.00133799988507366 0.00282448912315926]  Capacitance=[7.89543174552926e-09 -1.85986777702161e-09 -1.7901190036642e-09;-1.85986777702161e-09 7.82540023894543e-09 -1.8957321828871e-09;-1.7901190036642e-09 -1.8957321828871e-09 7.91264394645417e-09]  x1=[143.075564008337 4022.40983924515 4025.83828253699;314.159265358979 314.159265358979 314.159265358979;0.976622220327449 -0.499722028604549 -2.07067057833389]  x2=[143.076332660615 4022.35324504068 4025.78166275665;314.159265358979 314.159265358979 314.159265358979;0.976623537201318 -0.499732503588856 -2.07068098678354]  x3=[0.126929394779951 9.57242062978139 9.65914879134469;314.159265358979 314.159265358979 314.159265358979;0.957570105846559 -0.498000360119259 -2.06898460815199]  x4=[0.123292403060627 10.8973778891244 10.9854247653321;314.159265358979 314.159265358979 314.159265358979;0.996023935139009 -0.501401433169646 -2.07232022883204]  x5=6.70710350311308e-07  V1=ones(3,3)  V2=ones(3,3)  I1=ones(3,3)  I2=ones(3,3)  nHarmo=1  Measurements=None  Decoupling=off  VsMag0=0  VrMag0=0  VsAngle0=0  VrAngle0=0  IsMag0=0  IrMag0=0  IsAngle0=0  IrAngle0=0
      settings: SourceProductBaseCode=PS
  Line 70 : spsDistributedParametersLineLib/Distributed Parameters Line  Phases=3  Length=0.50001  Frequency=50  Resistance=[0.646656091154803 0.0486237908083191 0.0486712220507153;0.0486237908083191 0.646561225344642 0.0486237934466192;0.0486712220507153 0.0486237934466192 0.646656091154803]  Inductance=[0.00282448912315926 0.00133270803418135 0.00132951476746136;0.00133270803418135 0.00282479813276775 0.00133799988507366;0.00132951476746136 0.00133799988507366 0.00282448912315926]  Capacitance=[7.89543174552926e-09 -1.85986777702161e-09 -1.7901190036642e-09;-1.85986777702161e-09 7.82540023894543e-09 -1.8957321828871e-09;-1.7901190036642e-09 -1.8957321828871e-09 7.91264394645417e-09]  x1=[115.123155086607 8164.85933615105 8165.42238197054;314.159265358979 314.159265358979 314.159265358979;0.878987872954273 -0.343268528325121 -1.91479580828552]  x2=[119.810283207196 7427.11552101013 7428.22674768885;314.159265358979 314.159265358979 314.159265358979;0.898808346363083 -0.358191810957328 -1.92967358374592]  x3=[5.65929543767566 1945.45525337157 1948.93886709289;314.159265358979 314.159265358979 314.159265358979;0.197648027724856 2.27587349204616 0.707191894875792]  x4=[5.50261664142312 1980.06320803114 1983.87129167289;314.159265358979 314.159265358979 314.159265358979;-2.96773242883251 -0.855853906510163 -2.42452734968235]  x5=2.3957842710327e-06  V1=ones(3,3)  V2=ones(3,3)  I1=ones(3,3)  I2=ones(3,3)  nHarmo=1  Measurements=None  Decoupling=off  VsMag0=0  VrMag0=0  VsAngle0=0  VrAngle0=0  IsMag0=0  IrMag0=0  IsAngle0=0  IrAngle0=0
      settings: SourceProductBaseCode=PS
  Line 71 : spsDistributedParametersLineLib/Distributed Parameters Line  Phases=3  Length=0.17  Frequency=50  Resistance=[0.646656091154803 0.0486237908083191 0.0486712220507153;0.0486237908083191 0.646561225344642 0.0486237934466192;0.0486712220507153 0.0486237934466192 0.646656091154803]  Inductance=[0.00282448912315926 0.00133270803418135 0.00132951476746136;0.00133270803418135 0.00282479813276775 0.00133799988507366;0.00132951476746136 0.00133799988507366 0.00282448912315926]  Capacitance=[7.89543174552926e-09 -1.85986777702161e-09 -1.7901190036642e-09;-1.85986777702161e-09 7.82540023894543e-09 -1.8957321828871e-09;-1.7901190036642e-09 -1.8957321828871e-09 7.91264394645417e-09]  x1=[115.123155086607 8164.85933615105 8165.42238197054;314.159265358979 314.159265358979 314.159265358979;0.879484632237764 -0.342873885700548 -1.91440078998911]  x2=[115.123886015032 8164.75462407686 8165.31788788617;314.159265358979 314.159265358979 314.159265358979;0.879486572460853 -0.342875331343956 -1.91440219545571]  x3=[0.102215976640722 20.0859914261756 20.2466197141815;314.159265358979 314.159265358979 314.159265358979;0.861472536862444 -0.321634128036532 -1.89333553598471]  x4=[0.0991136090902076 21.4718761547251 21.633122391433;314.159265358979 314.159265358979 314.159265358979;0.897802648955465 -0.362940696719559 -1.93431409376242]  x5=8.14550361143895e-07  V1=ones(3,3)  V2=ones(3,3)  I1=ones(3,3)  I2=ones(3,3)  nHarmo=1  Measurements=None  Decoupling=off  VsMag0=0  VrMag0=0  VsAngle0=0  VrAngle0=0  IsMag0=0  IrMag0=0  IsAngle0=0  IrAngle0=0
      settings: SourceProductBaseCode=PS
  Line 72 : spsDistributedParametersLineLib/Distributed Parameters Line  Phases=3  Length=0.27999  Frequency=50  Resistance=[0.646656091154803 0.0486237908083191 0.0486712220507153;0.0486237908083191 0.646561225344642 0.0486237934466192;0.0486712220507153 0.0486237934466192 0.646656091154803]  Inductance=[0.00282448912315926 0.00133270803418135 0.00132951476746136;0.00133270803418135 0.00282479813276775 0.00133799988507366;0.00132951476746136 0.00133799988507366 0.00282448912315926]  Capacitance=[7.89543174552926e-09 -1.85986777702161e-09 -1.7901190036642e-09;-1.85986777702161e-09 7.82540023894543e-09 -1.8957321828871e-09;-1.7901190036642e-09 -1.8957321828871e-09 7.91264394645417e-09]  x1=[112.518309621137 8578.8315378858 8579.08319534746;314.159265358979 314.159265358979 314.159265358979;0.867498298180719 -0.335768433806014 -1.90731671639912]  x2=[115.123155086607 8164.85933615105 8165.42238197054;314.159265358979 314.159265358979 314.159265358979;0.879319065880406 -0.343005417297399 -1.91453244679473]  x3=[5.66105211503433 1945.75608155197 1949.23498981079;314.159265358979 314.159265358979 314.159265358979;0.197480208921857 2.27578680968852 0.707104087750774]  x4=[5.50719277902588 1982.70308020387 1986.52843667059;314.159265358979 314.159265358979 314.159265358979;-2.96671739653348 -0.855012509709891 -2.42368616933668]  x5=1.341564444804e-06  V1=ones(3,3)  V2=ones(3,3)  I1=ones(3,3)  I2=ones(3,3)  nHarmo=1  Measurements=None  Decoupling=off  VsMag0=0  VrMag0=0  VsAngle0=0  VrAngle0=0  IsMag0=0  IrMag0=0  IsAngle0=0  IrAngle0=0
      settings: SourceProductBaseCode=PS
  Line 73 : spsDistributedParametersLineLib/Distributed Parameters Line  Phases=3  Length=0.01  Frequency=50  Resistance=[0.646656091154803 0.0486237908083191 0.0486712220507153;0.0486237908083191 0.646561225344642 0.0486237934466192;0.0486712220507153 0.0486237934466192 0.646656091154803]  Inductance=[0.00282448912315926 0.00133270803418135 0.00132951476746136;0.00133270803418135 0.00282479813276775 0.00133799988507366;0.00132951476746136 0.00133799988507366 0.00282448912315926]  Capacitance=[7.89543174552926e-09 -1.85986777702161e-09 -1.7901190036642e-09;-1.85986777702161e-09 7.82540023894543e-09 -1.8957321828871e-09;-1.7901190036642e-09 -1.8957321828871e-09 7.91264394645417e-09]  x1=[112.425573496477 8593.62466553572 8593.86515579965;314.159265358979 314.159265358979 314.159265358979;0.867472406269434 -0.335199988850362 -1.90674867521682]  x2=[112.518309621137 8578.8315378858 8579.08319534746;314.159265358979 314.159265358979 314.159265358979;0.867904710225659 -0.335445566128645 -1.90699354137459]  x3=[5.66151535519486 1946.12393814634 1949.6062518653;314.159265358979 314.159265358979 314.159265358979;0.197872112294189 2.27609705013857 0.707414618485122]  x4=[5.50868704919448 1983.94930853641 1987.78639417934;314.159265358979 314.159265358979 314.159265358979;-2.96588792604415 -0.854356545835665 -2.42302959357717]  x5=4.79147271261115e-08  V1=ones(3,3)  V2=ones(3,3)  I1=ones(3,3)  I2=ones(3,3)  nHarmo=1  Measurements=None  Decoupling=off  VsMag0=0  VrMag0=0  VsAngle0=0  VrAngle0=0  IsMag0=0  IrMag0=0  IsAngle0=0  IrAngle0=0
      settings: SourceProductBaseCode=PS
  Line 74 : spsDistributedParametersLineLib/Distributed Parameters Line  Phases=3  Length=0.04  Frequency=50  Resistance=[0.646656091154803 0.0486237908083191 0.0486712220507153;0.0486237908083191 0.646561225344642 0.0486237934466192;0.0486712220507153 0.0486237934466192 0.646656091154803]  Inductance=[0.00282448912315926 0.00133270803418135 0.00132951476746136;0.00133270803418135 0.00282479813276775 0.00133799988507366;0.00132951476746136 0.00133799988507366 0.00282448912315926]  Capacitance=[7.89543174552926e-09 -1.85986777702161e-09 -1.7901190036642e-09;-1.85986777702161e-09 7.82540023894543e-09 -1.8957321828871e-09;-1.7901190036642e-09 -1.8957321828871e-09 7.91264394645417e-09]  x1=[112.054839719995 8652.80230219014 8652.99809410196;314.159265358979 314.159265358979 314.159265358979;0.865690879831667 -0.334261950826533 -1.90581348498209]  x2=[112.425573496477 8593.62466553572 8593.86515579965;314.159265358979 314.159265358979 314.159265358979;0.867427247703013 -0.335235864365459 -1.90678458488287]  x3=[5.66131485849074 1945.96015439627 1949.44093708067;314.159265358979 314.159265358979 314.159265358979;0.197766968485136 2.27601305879878 0.70733054505761]  x4=[5.50867004010656 1983.93371029367 1987.77064476418;314.159265358979 314.159265358979 314.159265358979;-2.96591790320163 -0.854380608412613 -2.42305368012341]  x5=1.91658908504446e-07  V1=ones(3,3)  V2=ones(3,3)  I1=ones(3,3)  I2=ones(3,3)  nHarmo=1  Measurements=None  Decoupling=off  VsMag0=0  VrMag0=0  VsAngle0=0  VrAngle0=0  IsMag0=0  IrMag0=0  IsAngle0=0  IrAngle0=0
      settings: SourceProductBaseCode=PS
  Line 8 : spsDistributedParametersLineLib/Distributed Parameters Line  Phases=3  Length=0.14997  Frequency=50  Resistance=[0.476003738225748 0.351747138225748 0.351747138225748;0.351747138225748 0.476003738225748 0.351747138225748;0.351747138225748 0.351747138225748 0.476003738225748]  Inductance=[0.000705954362986426 0.000459934243504405 0.000459934243504405;0.000459934243504405 0.000705954362986426 0.000459934243504405;0.000459934243504405 0.000459934243504405 0.000705954362986426]  Capacitance=[5.7561313269996e-07 -1.37543883484145e-07 -1.37543912800485e-07;-1.37543883484145e-07 5.75613027339387e-07 -1.37543875208088e-07;-1.37543912800485e-07 -1.37543875208088e-07 5.75613005057695e-07]  x1=[93.9426104286555 4022.79247710475 4026.33903366424;314.159265358979 314.159265358979 314.159265358979;1.13059216061929 -0.418513000554566 -1.98940943296175]  x2=[93.9426613733754 4022.77913803019 4026.32568282962;314.159265358979 314.159265358979 314.159265358979;1.13059090835728 -0.418514512855353 -1.98941094526249]  x3=[1.27492162844006 215.763128886871 215.953332291998;314.159265358979 314.159265358979 314.159265358979;1.12955011254571 -0.418429330176345 -1.98932576247769]  x4=[1.27492161114297 217.086889242063 217.27825969448;314.159265358979 314.159265358979 314.159265358979;1.13059089717599 -0.419219990074625 -1.99011642253847]  x5=3.31498451375949e-06  V1=ones(3,3)  V2=ones(3,3)  I1=ones(3,3)  I2=ones(3,3)  nHarmo=1  Measurements=None  Decoupling=off  VsMag0=0  VrMag0=0  VsAngle0=0  VrAngle0=0  IsMag0=0  IrMag0=0  IsAngle0=0  IrAngle0=0
      settings: SourceProductBaseCode=PS
  Line 9 : spsDistributedParametersLineLib/Distributed Parameters Line  Phases=3  Length=0.50001  Frequency=50  Resistance=[0.646656091154803 0.0486237908083191 0.0486712220507153;0.0486237908083191 0.646561225344642 0.0486237934466192;0.0486712220507153 0.0486237934466192 0.646656091154803]  Inductance=[0.00282448912315926 0.00133270803418135 0.00132951476746136;0.00133270803418135 0.00282479813276775 0.00133799988507366;0.00132951476746136 0.00133799988507366 0.00282448912315926]  Capacitance=[7.89543174552926e-09 -1.85986777702161e-09 -1.7901190036642e-09;-1.85986777702161e-09 7.82540023894543e-09 -1.8957321828871e-09;-1.7901190036642e-09 -1.8957321828871e-09 7.91264394645417e-09]  x1=[137.717423229215 4738.81854218925 4741.80718996898;314.159265358979 314.159265358979 314.159265358979;0.960848095670145 -0.45276042459361 -2.02390511830925]  x2=[143.075564008336 4022.40983924515 4025.83828253699;314.159265358979 314.159265358979 314.159265358979;0.976080272371824 -0.500152570661229 -2.07110153023612]  x3=[6.23928293110397 1949.38311058024 1952.86485500255;314.159265358979 314.159265358979 314.159265358979;0.19808860098192 2.27867017968104 0.710041987457268]  x4=[6.06551111480302 1970.02176332354 1973.6977108508;314.159265358979 314.159265358979 314.159265358979;-2.97168101932433 -0.858643035917579 -2.42726885640627]  x5=2.3957842710327e-06  V1=ones(3,3)  V2=ones(3,3)  I1=ones(3,3)  I2=ones(3,3)  nHarmo=1  Measurements=None  Decoupling=off  VsMag0=0  VrMag0=0  VsAngle0=0  VrAngle0=0  IsMag0=0  IrMag0=0  IsAngle0=0  IrAngle0=0
      settings: SourceProductBaseCode=PS
  Line im1 : spsDistributedParametersLineLib/Distributed Parameters Line  Phases=3  Length=1e-10  Frequency=50  Resistance=[0.646656091154803 0.0486237908083191 0.0486712220507153;0.0486237908083191 0.646561225344642 0.0486237934466192;0.0486712220507153 0.0486237934466192 0.646656091154803]  Inductance=[0.00282448912315926 0.00133270803418135 0.00132951476746136;0.00133270803418135 0.00282479813276775 0.00133799988507366;0.00132951476746136 0.00133799988507366 0.00282448912315926]  Capacitance=[7.89543174552926e-09 -1.85986777702161e-09 -1.7901190036642e-09;-1.85986777702161e-09 7.82540023894543e-09 -1.8957321828871e-09;-1.7901190036642e-09 -1.8957321828871e-09 7.91264394645417e-09]  x1=[159.41925430945 1994.46757360395 1998.0250826666;314.159265358979 314.159265358979 314.159265358979;1.01656994901145 -0.84612447869503 -2.41516984119514]  x2=[159.419254310559 1994.4675734855 1998.0250825481;314.159265358979 314.159265358979 314.159265358979;1.0165699490132 -0.846124478740392 -2.41516984124024]  x3=[6.18295277768854 1954.97427647394 1957.74049035222;314.159265358979 314.159265358979 314.159265358979;0.115896133208313 2.281591450617 0.713558487226471]  x4=[6.01378060787543 1965.12176921443 1967.98558277728;314.159265358979 314.159265358979 314.159265358979;-3.06223081619778 -0.859929003270297 -2.42796795116004]  x5=4.79147271261115e-16  V1=ones(3,3)  V2=ones(3,3)  I1=ones(3,3)  I2=ones(3,3)  nHarmo=1  Measurements=None  Decoupling=off  VsMag0=0  VrMag0=0  VsAngle0=0  VrAngle0=0  IsMag0=0  IrMag0=0  IsAngle0=0  IrAngle0=0
      settings: SourceProductBaseCode=PS
  Line im3 : spsDistributedParametersLineLib/Distributed Parameters Line  Phases=3  Length=1e-10  Frequency=50  Resistance=[0.646656091154803 0.0486237908083191 0.0486712220507153;0.0486237908083191 0.646561225344642 0.0486237934466192;0.0486712220507153 0.0486237934466192 0.646656091154803]  Inductance=[0.00282448912315926 0.00133270803418135 0.00132951476746136;0.00133270803418135 0.00282479813276775 0.00133799988507366;0.00132951476746136 0.00133799988507366 0.00282448912315926]  Capacitance=[7.89543174552926e-09 -1.85986777702161e-09 -1.7901190036642e-09;-1.85986777702161e-09 7.82540023894543e-09 -1.8957321828871e-09;-1.7901190036642e-09 -1.8957321828871e-09 7.91264394645417e-09]  x1=[134.198860361112 5216.25494947947 5218.9203857818;314.159265358979 314.159265358979 314.159265358979;0.950882611545954 -0.428046933589352 -1.99928247256923]  x2=[134.198860362037 5216.25494933431 5218.9203856369;314.159265358979 314.159265358979 314.159265358979;0.950882611547679 -0.428046933595978 -1.99928247257589]  x3=[5.15166733370893 1950.19322008355 1952.42666641159;314.159265358979 314.159265358979 314.159265358979;0.0513106684046658 2.27833102515696 0.711626843786856]  x4=[5.01374377617265 1974.30598521536 1976.78062209815;314.159265358979 314.159265358979 314.159265358979;-3.12748743736964 -0.857591139671783 -2.4243132238833]  x5=4.79147271261115e-16  V1=ones(3,3)  V2=ones(3,3)  I1=ones(3,3)  I2=ones(3,3)  nHarmo=1  Measurements=None  Decoupling=off  VsMag0=0  VrMag0=0  VsAngle0=0  VrAngle0=0  IsMag0=0  IrMag0=0  IsAngle0=0  IrAngle0=0
      settings: SourceProductBaseCode=PS
  Load 1 : spsThreePhaseSeriesRLCLoadLib/Three-Phase Series RLC Load  LConnTagsString=A|B|C  Configuration=Delta  NominalVoltage=11000  Vabc=[1e3 1e3 1e3]  Vabcp=[1e3 1e3 1e3]  NominalFrequency=50  UnbalancedPower=off  ActivePower=21338.9466  InductivePower=15261.1898  CapacitivePower=0  Pabc=[10e3 9e3 11e3]  QLabc=[100 90 110]  QCabc=[100 90 110]  Pabcp=[10e3 9e3 11e3]  QLabcp=[100 90 110]  QCabcp=[100 90 110]  Measurements=None  LoadType=constant Z
  Load 2 : spsThreePhaseSeriesRLCLoadLib/Three-Phase Series RLC Load  LConnTagsString=A|B|C  Configuration=Delta  NominalVoltage=11000  Vabc=[1e3 1e3 1e3]  Vabcp=[1e3 1e3 1e3]  NominalFrequency=50  UnbalancedPower=off  ActivePower=21200.9244  InductivePower=15700.0686  CapacitivePower=0  Pabc=[10e3 9e3 11e3]  QLabc=[100 90 110]  QCabc=[100 90 110]  Pabcp=[10e3 9e3 11e3]  QLabcp=[100 90 110]  QCabcp=[100 90 110]  Measurements=None  LoadType=constant Z
  Load 3 : spsThreePhaseSeriesRLCLoadLib/Three-Phase Series RLC Load  LConnTagsString=A|B|C  Configuration=Delta  NominalVoltage=11000  Vabc=[1e3 1e3 1e3]  Vabcp=[1e3 1e3 1e3]  NominalFrequency=50  UnbalancedPower=off  ActivePower=27934.5568  InductivePower=8494.123  CapacitivePower=0  Pabc=[10e3 9e3 11e3]  QLabc=[100 90 110]  QCabc=[100 90 110]  Pabcp=[10e3 9e3 11e3]  QLabcp=[100 90 110]  QCabcp=[100 90 110]  Measurements=None  LoadType=constant Z
  Load 4 : spsThreePhaseSeriesRLCLoadLib/Three-Phase Series RLC Load  LConnTagsString=A|B|C  Configuration=Delta  NominalVoltage=11000  Vabc=[1e3 1e3 1e3]  Vabcp=[1e3 1e3 1e3]  NominalFrequency=50  UnbalancedPower=off  ActivePower=187.8068  InductivePower=40.9242  CapacitivePower=0  Pabc=[10e3 9e3 11e3]  QLabc=[100 90 110]  QCabc=[100 90 110]  Pabcp=[10e3 9e3 11e3]  QLabcp=[100 90 110]  QCabcp=[100 90 110]  Measurements=None  LoadType=constant Z
  Load 5 : spsThreePhaseSeriesRLCLoadLib/Three-Phase Series RLC Load  LConnTagsString=A|B|C  Configuration=Delta  NominalVoltage=11000  Vabc=[1e3 1e3 1e3]  Vabcp=[1e3 1e3 1e3]  NominalFrequency=50  UnbalancedPower=off  ActivePower=3781.4291  InductivePower=1551.1354  CapacitivePower=0  Pabc=[10e3 9e3 11e3]  QLabc=[100 90 110]  QCabc=[100 90 110]  Pabcp=[10e3 9e3 11e3]  QLabcp=[100 90 110]  QCabcp=[100 90 110]  Measurements=None  LoadType=constant Z
  Load 8041 : spsThreePhaseSeriesRLCLoadLib/Three-Phase Series RLC Load  LConnTagsString=A|B|C  Configuration=Delta  NominalVoltage=11000  Vabc=[1e3 1e3 1e3]  Vabcp=[1e3 1e3 1e3]  NominalFrequency=50  UnbalancedPower=off  ActivePower=11589.9741  InductivePower=7378.5065  CapacitivePower=0  Pabc=[10e3 9e3 11e3]  QLabc=[100 90 110]  QCabc=[100 90 110]  Pabcp=[10e3 9e3 11e3]  QLabcp=[100 90 110]  QCabcp=[100 90 110]  Measurements=None  LoadType=constant Z
  Load 8173 : spsThreePhaseSeriesRLCLoadLib/Three-Phase Series RLC Load  LConnTagsString=A|B|C  Configuration=Delta  NominalVoltage=11000  Vabc=[1e3 1e3 1e3]  Vabcp=[1e3 1e3 1e3]  NominalFrequency=50  UnbalancedPower=off  ActivePower=14077.2749  InductivePower=10251.6352  CapacitivePower=0  Pabc=[10e3 9e3 11e3]  QLabc=[100 90 110]  QCabc=[100 90 110]  Pabcp=[10e3 9e3 11e3]  QLabcp=[100 90 110]  QCabcp=[100 90 110]  Measurements=None  LoadType=constant Z
  Load 8287 : spsThreePhaseSeriesRLCLoadLib/Three-Phase Series RLC Load  LConnTagsString=A|B|C  Configuration=Delta  NominalVoltage=11000  Vabc=[1e3 1e3 1e3]  Vabcp=[1e3 1e3 1e3]  NominalFrequency=50  UnbalancedPower=off  ActivePower=17265.4544  InductivePower=7182.7775  CapacitivePower=0  Pabc=[10e3 9e3 11e3]  QLabc=[100 90 110]  QCabc=[100 90 110]  Pabcp=[10e3 9e3 11e3]  QLabcp=[100 90 110]  QCabcp=[100 90 110]  Measurements=None  LoadType=constant Z
  Load 8293 : spsThreePhaseSeriesRLCLoadLib/Three-Phase Series RLC Load  LConnTagsString=A|B|C  Configuration=Delta  NominalVoltage=11000  Vabc=[1e3 1e3 1e3]  Vabcp=[1e3 1e3 1e3]  NominalFrequency=50  UnbalancedPower=off  ActivePower=3530.6466  InductivePower=1992.4739  CapacitivePower=0  Pabc=[10e3 9e3 11e3]  QLabc=[100 90 110]  QCabc=[100 90 110]  Pabcp=[10e3 9e3 11e3]  QLabcp=[100 90 110]  QCabcp=[100 90 110]  Measurements=None  LoadType=constant Z
  Load 8424 : spsThreePhaseSeriesRLCLoadLib/Three-Phase Series RLC Load  LConnTagsString=A|B|C  Configuration=Delta  NominalVoltage=11000  Vabc=[1e3 1e3 1e3]  Vabcp=[1e3 1e3 1e3]  NominalFrequency=50  UnbalancedPower=off  ActivePower=7882.3727  InductivePower=625.1347  CapacitivePower=0  Pabc=[10e3 9e3 11e3]  QLabc=[100 90 110]  QCabc=[100 90 110]  Pabcp=[10e3 9e3 11e3]  QLabcp=[100 90 110]  QCabcp=[100 90 110]  Measurements=None  LoadType=constant Z
  Load 8485 : spsThreePhaseSeriesRLCLoadLib/Three-Phase Series RLC Load  LConnTagsString=A|B|C  Configuration=Delta  NominalVoltage=11000  Vabc=[1e3 1e3 1e3]  Vabcp=[1e3 1e3 1e3]  NominalFrequency=50  UnbalancedPower=off  ActivePower=29844.4282  InductivePower=11288.3714  CapacitivePower=0  Pabc=[10e3 9e3 11e3]  QLabc=[100 90 110]  QCabc=[100 90 110]  Pabcp=[10e3 9e3 11e3]  QLabcp=[100 90 110]  QCabcp=[100 90 110]  Measurements=None  LoadType=constant Z
  Load 8551 : spsThreePhaseSeriesRLCLoadLib/Three-Phase Series RLC Load  LConnTagsString=A|B|C  Configuration=Delta  NominalVoltage=11000  Vabc=[1e3 1e3 1e3]  Vabcp=[1e3 1e3 1e3]  NominalFrequency=50  UnbalancedPower=off  ActivePower=10178.6282  InductivePower=3222.3399  CapacitivePower=0  Pabc=[10e3 9e3 11e3]  QLabc=[100 90 110]  QCabc=[100 90 110]  Pabcp=[10e3 9e3 11e3]  QLabcp=[100 90 110]  QCabcp=[100 90 110]  Measurements=None  LoadType=constant Z
  Load 8605 : spsThreePhaseSeriesRLCLoadLib/Three-Phase Series RLC Load  LConnTagsString=A|B|C  Configuration=Delta  NominalVoltage=11000  Vabc=[1e3 1e3 1e3]  Vabcp=[1e3 1e3 1e3]  NominalFrequency=50  UnbalancedPower=off  ActivePower=108.5393  InductivePower=42.0469  CapacitivePower=0  Pabc=[10e3 9e3 11e3]  QLabc=[100 90 110]  QCabc=[100 90 110]  Pabcp=[10e3 9e3 11e3]  QLabcp=[100 90 110]  QCabcp=[100 90 110]  Measurements=None  LoadType=constant Z
  Load 8733 : spsThreePhaseSeriesRLCLoadLib/Three-Phase Series RLC Load  LConnTagsString=A|B|C  Configuration=Delta  NominalVoltage=11000  Vabc=[1e3 1e3 1e3]  Vabcp=[1e3 1e3 1e3]  NominalFrequency=50  UnbalancedPower=off  ActivePower=2766.9291  InductivePower=1648.384  CapacitivePower=0  Pabc=[10e3 9e3 11e3]  QLabc=[100 90 110]  QCabc=[100 90 110]  Pabcp=[10e3 9e3 11e3]  QLabcp=[100 90 110]  QCabcp=[100 90 110]  Measurements=None  LoadType=constant Z
  Load 8737 : spsThreePhaseSeriesRLCLoadLib/Three-Phase Series RLC Load  LConnTagsString=A|B|C  Configuration=Delta  NominalVoltage=11000  Vabc=[1e3 1e3 1e3]  Vabcp=[1e3 1e3 1e3]  NominalFrequency=50  UnbalancedPower=off  ActivePower=12961.3673  InductivePower=6071.527  CapacitivePower=0  Pabc=[10e3 9e3 11e3]  QLabc=[100 90 110]  QCabc=[100 90 110]  Pabcp=[10e3 9e3 11e3]  QLabcp=[100 90 110]  QCabcp=[100 90 110]  Measurements=None  LoadType=constant Z
  R1 : spsThreePhaseVIMeasurementLib/Three-Phase V-I Measurement  VoltageMeasurement=phase-to-ground  SetLabelV=off  LabelV=Vabc  Vpu=off  VpuLL=off  CurrentMeasurement=yes  SetLabelI=off  LabelI=Iabc  Ipu=off  Pbase=100e6  Vbase=500e3  OutputType=Complex  PhasorSimulation=on  PSBequivalent=0
  R2 : spsThreePhaseVIMeasurementLib/Three-Phase V-I Measurement  VoltageMeasurement=phase-to-ground  SetLabelV=off  LabelV=Vabc  Vpu=off  VpuLL=off  CurrentMeasurement=yes  SetLabelI=off  LabelI=Iabc  Ipu=off  Pbase=100e6  Vbase=500e3  OutputType=Complex  PhasorSimulation=on  PSBequivalent=0
  R5 : spsThreePhaseVIMeasurementLib/Three-Phase V-I Measurement  VoltageMeasurement=phase-to-ground  SetLabelV=off  LabelV=Vabc  Vpu=off  VpuLL=off  CurrentMeasurement=yes  SetLabelI=off  LabelI=Iabc  Ipu=off  Pbase=100e6  Vbase=500e3  OutputType=Complex  PhasorSimulation=on  PSBequivalent=0
  Scope R1 : Scope  NumInputPorts=2
  Scope R2 : Scope  NumInputPorts=2
  Scope R5 : Scope  NumInputPorts=2
  Source PC1_TT2 : spsThreePhaseSourceLib/Three-Phase Source  InternalConnection=Yn  VoltagePhases=off  Voltage=10000  PhaseAngle=0  Voltage_phases=[25e3 25e3 25e3]/sqrt(3)  PhaseAngles_phases=[0 -120 +120]  Frequency=50  NonIdealSource=on  SpecifyImpedance=off  Resistance=0.14  Inductance=0.0031831  ShortCircuitLevel=100e6  BaseVoltage=25e3  XRratio=7  BusType=swing  Pref=10e3  Qref=0  Prefabc=[10e3, 10e3, 10e3]  Qrefabc=[0, 0, 0]  Qmin=-inf  Qmax=inf
  Source Zn : spsSeriesRLCBranchLib/Series RLC Branch  LConnTagsString=__new0  RConnTagsString=__new0  BranchType=RL  Resistance=0.001  Inductance=3.1831e-06  SetiL0=off  InitialCurrent=0  Capacitance=0  Setx0=off  InitialVoltage=0  Measurements=None
  powergui : spspowerguiLib/powergui  Priority=1  SimulationMode=Phasor  SampleTime=50e-6  frequency=50  Iterations=50  frequencyindice=50  Pbase=100e6  ErrMax=1e-4  UnitsV=kV  UnitsW=MW  buscounter=0  FunctionMessages=off  echomessages=off  EnableUseOfTLC=off  CurrentSourceSwitches=off  DisableSnubberDevices=off  DisableRonSwitches=off  DisableVfSwitches=off  DisplayEquations=off  AutomaticDiscreteSolvers=off  SolverType=Tustin/Backward Euler (TBE)  Interpol=off  ExternalGateDelay=off  methode=off  Ts=10  x0status=blocks  SPID=off  SwTol=0  HookPort=off  NonlinearTolerance=1e-4  nMaxIteration=100  ContinueOnMaxIteration=off  RestoreLinks=warning  ResistiveCurrentMeasurement=off  Frange=[0:2:500]  Ylog=off  Xlog=on  ShowGrid=off  save=off  variable=ZData  structure=0  ZoomFFT=off  StartTime=0.0  cycles=1  DisplayStyle=1  fundamental=60  FreqAxis=off  MaxFrequency=1000  frequencyindicesteady=1  RmsSteady=1  display=off
  wires:
  R5/2 -> Scope R5/2
  R2/1 -> Scope R2/1
  R5/1 -> Scope R5/1
  R2/2 -> Scope R2/2
  R1/2 -> Scope R1/2
  R1/1 -> Scope R1/1
  connections:
  Source Zn/RConn1 -- Source PC1_TT2/LConn1
  Source Zn/LConn1 -- Ground/LConn1
  Line im3/RConn1 -- Line 13/LConn1
  Line im3/RConn2 -- Line 13/LConn2
  Line im3/RConn3 -- Line 13/LConn3
  Load 8733/LConn1 -- Line 63/RConn1
  Load 8733/LConn2 -- Line 63/RConn2
  Load 8733/LConn3 -- Line 63/RConn3
  Line 66/LConn1 -- Line 65/LConn1 -- Line 67/RConn1
  Line 66/LConn2 -- Line 65/LConn2 -- Line 67/RConn2
  Line 66/LConn3 -- Line 65/LConn3 -- Line 67/RConn3
  Line im1/LConn1 -- R1/RConn1
  Line im1/LConn2 -- R1/RConn2
  Line im1/LConn3 -- R1/RConn3
  Line 71/LConn1 -- Line 70/LConn1 -- Line 72/RConn1
  Line 71/LConn2 -- Line 70/LConn2 -- Line 72/RConn2
  Line 71/LConn3 -- Line 70/LConn3 -- Line 72/RConn3
  Line 8/RConn1 -- Load 2/LConn1
  Line 8/RConn2 -- Load 2/LConn2
  Line 8/RConn3 -- Load 2/LConn3
  Line 5/LConn1 -- Line 4/LConn1 -- Line 6/RConn1
  Line 5/LConn2 -- Line 4/LConn2 -- Line 6/RConn2
  Line 5/LConn3 -- Line 4/LConn3 -- Line 6/RConn3
  Line 56/LConn1 -- Line 55/LConn1 -- Line 54/RConn1
  Line 56/LConn2 -- Line 55/LConn2 -- Line 54/RConn2
  Line 56/LConn3 -- Line 55/LConn3 -- Line 54/RConn3
  Load 5/LConn1 -- Line 2/RConn1
  Load 5/LConn2 -- Line 2/RConn2
  Load 5/LConn3 -- Line 2/RConn3
  Line 74/LConn1 -- R2/RConn1
  Line 74/LConn2 -- R2/RConn2
  Line 74/LConn3 -- R2/RConn3
  Line 7/RConn1 -- Line 8/LConn1
  Line 7/RConn2 -- Line 8/LConn2
  Line 7/RConn3 -- Line 8/LConn3
  Line 72/LConn1 -- Line 73/RConn1
  Line 72/LConn2 -- Line 73/RConn2
  Line 72/LConn3 -- Line 73/RConn3
  Line 58/RConn1 -- Load 8551/LConn1
  Line 58/RConn2 -- Load 8551/LConn2
  Line 58/RConn3 -- Load 8551/LConn3
  Line 49/LConn1 -- Line 48/LConn1 -- Line 47/RConn1
  Line 49/LConn2 -- Line 48/LConn2 -- Line 47/RConn2
  Line 49/LConn3 -- Line 48/LConn3 -- Line 47/RConn3
  Line 10/RConn1 -- Load 1/LConn1
  Line 10/RConn2 -- Load 1/LConn2
  Line 10/RConn3 -- Load 1/LConn3
  Line 69/RConn1 -- Load 8287/LConn1
  Line 69/RConn2 -- Load 8287/LConn2
  Line 69/RConn3 -- Load 8287/LConn3
  Line 62/RConn1 -- R5/LConn1
  Line 62/RConn2 -- R5/LConn2
  Line 62/RConn3 -- R5/LConn3
  Line 12/LConn1 -- Line 13/RConn1
  Line 12/LConn2 -- Line 13/RConn2
  Line 12/LConn3 -- Line 13/RConn3
  Load 3/LConn1 -- Line 3/LConn1 -- Line 4/RConn1
  Load 3/LConn2 -- Line 3/LConn2 -- Line 4/RConn2
  Load 3/LConn3 -- Line 3/LConn3 -- Line 4/RConn3
  Line 51/RConn1 -- Line 50/LConn1
  Line 51/RConn2 -- Line 50/LConn2
  Line 51/RConn3 -- Line 50/LConn3
  Line 7/LConn1 -- Line 6/LConn1 -- Line 9/RConn1
  Line 7/LConn2 -- Line 6/LConn2 -- Line 9/RConn2
  Line 7/LConn3 -- Line 6/LConn3 -- Line 9/RConn3
  Line im3/LConn1 -- R5/RConn1
  Line im3/LConn2 -- R5/RConn2
  Line im3/LConn3 -- R5/RConn3
  Line 66/RConn1 -- Load 8605/LConn1
  Line 66/RConn2 -- Load 8605/LConn2
  Line 66/RConn3 -- Load 8605/LConn3
  Line 1/RConn1 -- R1/LConn1
  Line 1/RConn2 -- R1/LConn2
  Line 1/RConn3 -- R1/LConn3
  Line 44/LConn1 -- Line 45/RConn1
  Line 44/LConn2 -- Line 45/RConn2
  Line 44/LConn3 -- Line 45/RConn3
  Load 8485/LConn1 -- Line 64/LConn1 -- Line 65/RConn1
  Load 8485/LConn2 -- Line 64/LConn2 -- Line 65/RConn2
  Load 8485/LConn3 -- Line 64/LConn3 -- Line 65/RConn3
  Line 55/RConn1 -- Load 8424/LConn1
  Line 55/RConn2 -- Load 8424/LConn2
  Line 55/RConn3 -- Load 8424/LConn3
  Line 68/LConn1 -- Line 67/LConn1 -- Line 70/RConn1
  Line 68/LConn2 -- Line 67/LConn2 -- Line 70/RConn2
  Line 68/LConn3 -- Line 67/LConn3 -- Line 70/RConn3
  Line 68/RConn1 -- Line 69/LConn1
  Line 68/RConn2 -- Line 69/LConn2
  Line 68/RConn3 -- Line 69/LConn3
  Source PC1_TT2/RConn1 -- R2/LConn1
  Source PC1_TT2/RConn2 -- R2/LConn2
  Source PC1_TT2/RConn3 -- R2/LConn3
  Line 11/LConn1 -- Line 12/RConn1
  Line 11/LConn2 -- Line 12/RConn2
  Line 11/LConn3 -- Line 12/RConn3
  Line 52/LConn1 -- Line 51/LConn1 -- Line 53/RConn1
  Line 52/LConn2 -- Line 51/LConn2 -- Line 53/RConn2
  Line 52/LConn3 -- Line 51/LConn3 -- Line 53/RConn3
  Line 5/RConn1 -- Load 4/LConn1
  Line 5/RConn2 -- Load 4/LConn2
  Line 5/RConn3 -- Load 4/LConn3
  Load 8737/LConn1 -- Line 52/RConn1
  Load 8737/LConn2 -- Line 52/RConn2
  Load 8737/LConn3 -- Line 52/RConn3
  Line 2/LConn1 -- Line 1/LConn1 -- Line 3/RConn1
  Line 2/LConn2 -- Line 1/LConn2 -- Line 3/RConn2
  Line 2/LConn3 -- Line 1/LConn3 -- Line 3/RConn3
  Line 73/LConn1 -- Line 74/RConn1
  Line 73/LConn2 -- Line 74/RConn2
  Line 73/LConn3 -- Line 74/RConn3
  Line 63/LConn1 -- Line 62/LConn1 -- Line 64/RConn1
  Line 63/LConn2 -- Line 62/LConn2 -- Line 64/RConn2
  Line 63/LConn3 -- Line 62/LConn3 -- Line 64/RConn3
  Line 54/LConn1 -- Line 53/LConn1 -- Line 59/RConn1
  Line 54/LConn2 -- Line 53/LConn2 -- Line 59/RConn2
  Line 54/LConn3 -- Line 53/LConn3 -- Line 59/RConn3
  Line 59/LConn1 -- Line 60/LConn1 -- Line im1/RConn1
  Line 59/LConn2 -- Line 60/LConn2 -- Line im1/RConn2
  Line 59/LConn3 -- Line 60/LConn3 -- Line im1/RConn3
  Line 46/RConn1 -- Line 47/LConn1
  Line 46/RConn2 -- Line 47/LConn2
  Line 46/RConn3 -- Line 47/LConn3
  Line 58/LConn1 -- Line 57/LConn1 -- Line 56/RConn1
  Line 58/LConn2 -- Line 57/LConn2 -- Line 56/RConn2
  Line 58/LConn3 -- Line 57/LConn3 -- Line 56/RConn3
  Line 10/LConn1 -- Line 9/LConn1 -- Line 11/RConn1
  Line 10/LConn2 -- Line 9/LConn2 -- Line 11/RConn2
  Line 10/LConn3 -- Line 9/LConn3 -- Line 11/RConn3
  Line 71/RConn1 -- Load 8041/LConn1
  Line 71/RConn2 -- Load 8041/LConn2
  Line 71/RConn3 -- Load 8041/LConn3
  Line 46/LConn1 -- Load 8173/LConn1 -- Line 50/RConn1 -- Line 45/LConn1
  Line 46/LConn2 -- Load 8173/LConn2 -- Line 50/RConn2 -- Line 45/LConn2
  Line 46/LConn3 -- Load 8173/LConn3 -- Line 50/RConn3 -- Line 45/LConn3
  Line 57/RConn1 -- Load 8293/LConn1
  Line 57/RConn2 -- Load 8293/LConn2
  Line 57/RConn3 -- Load 8293/LConn3
  Line 60/RConn1 -- Line 61/LConn1
  Line 60/RConn2 -- Line 61/LConn2
  Line 60/RConn3 -- Line 61/LConn3
